simulink library "ammclib_bam_S32K3xx"  (R2016a)
(part 26 of 50)

      | text(tX,tY, 'AMCLIB_FluxEstimAB_FLT', 'horizontalAlignment', 'center');
      | if showStates == 2
      |   color('red');
      |   text(tX,tY - 20, ['debugging mode' char(13) char(10) '(limited performance)'], 'horizontalAlignment', 'center');
      | end
  AMCLIB_SpeedLoop_FLT : Subsystem  StartFcn=|  TreatAsAtomicUnit=on  mask(AMCLIB_SpeedLoop_FLT){showStates=Hide (faster execution), resetStatesEnable=Pre-set according to the first set of inputs after reset, showDebugOutputs=Hide, fltState_Out_showOutput=off, SampleTime=-1, wf0=30, wksi=1, J=1.6e-5, Kt=0.067, lambdaW=0.9, ramprpm=6, mechspeed=3000, polepairs=1, autoCalcEn=on, fltLambdaW=0, fltPropGainQ=0, fltIntegGainQ=0, fltLowerLimitQ=0, fltUpperLimitQ=0, fltRampUp=0, fltRampDown=0, SampleTime_1=NaN}
      | ts=get_param(gcb,'CompiledSampleTime');
      | if iscell(ts)
      |   ts=ts{1};
      |   if iscell(ts)
      |     ts=ts{1};
      |   end
      | end
      | ts=ts(1);
      | set_param(gcb,'SampleTime_1',num2str(ts));
      | p=Simulink.Mask.get(gcb);
      | hintText=p.getDialogControl('timeHint');
      | SampleTime=Simulink.data.evalinGlobal(bdroot,get_param(gcb,'SampleTime'));
      | p=Simulink.Mask.get(gcb);
      | autoCalcEn=get_param(gcb,'autoCalcEn');
      | if strcmp(autoCalcEn,'on')
      |   if SampleTime==-1
      |     hintText.Prompt='Caution: Implementation parameters depend on inherited sample time. Make sure that the sample time of the block''s inputs corresponds to the sampling period in the target application.';
      |   else
      |     hintText.Prompt='Caution: Implementation parameters depend on the sample time. Make sure that the simulation time step corresponds to the sampling period in the target application.';
      |   end
      |   SampleTime=ts;
      |   fltLambdaW_bkup=get_param(gcb,'fltLambdaW');
      |   fltPropGainQ_bkup=get_param(gcb,'fltPropGainQ');
      |   fltIntegGainQ_bkup=get_param(gcb,'fltIntegGainQ');
      |   fltLowerLimitQ_bkup=get_param(gcb,'fltLowerLimitQ');
      |   fltUpperLimitQ_bkup=get_param(gcb,'fltUpperLimitQ');
      |   fltRampUp_bkup=get_param(gcb,'fltRampUp');
      |   fltRampDown_bkup=get_param(gcb,'fltRampDown');
      |   wf0=Simulink.data.evalinGlobal(bdroot,get_param(gcb,'wf0'));
      |   wksi=Simulink.data.evalinGlobal(bdroot,get_param(gcb,'wksi'));
      |   J=Simulink.data.evalinGlobal(bdroot,get_param(gcb,'J'));
      |   Kt=Simulink.data.evalinGlobal(bdroot,get_param(gcb,'Kt'));
      |   lambdaW=Simulink.data.evalinGlobal(bdroot,get_param(gcb,'lambdaW'));
      |   ramprpm=Simulink.data.evalinGlobal(bdroot,get_param(gcb,'ramprpm'));
      |   mechspeed=Simulink.data.evalinGlobal(bdroot,get_param(gcb,'mechspeed'));
      |   polepairs=Simulink.data.evalinGlobal(bdroot,get_param(gcb,'polepairs'));
      |   if (wf0<=0)
      |     warning('Natural frequency f0 must be positive.');
      |   end
      |   if (wksi<=0)
      |     warning('Current loop attenuation must be positive.');
      |   end
      |   if (wksi>1)
      |     warning('Current loop attenuation must not exceed 1.');
      |   end
      |   if (J<=0)
      |     warning('Moment of inertia J must be positive.');
      |   end
      |   if (Kt<=0)
      |     warning('Torque constant Kt must be positive.');
      |   end
      |   if (lambdaW<0)
      |     warning('MA filter smoothing factor must be in the range 0..1.');
      |   end
      |   if (lambdaW>1)
      |     warning('MA filter smoothing factor must be in the range 0..1.');
      |   end
      |   if (mechspeed<=0)
      |     warning('Max. speed must be positive.');
      |   end
      |   if (polepairs<1)
      |     warning('Number of pole pairs must be a natural number (1, 2, 3, ...).');
      |   end
      |   if (round(polepairs)~=polepairs)
      |     warning('Number of pole pairs must be a natural number (1, 2, 3, ...).');
      |   end
      |   w0=6.283185307179586*wf0;
      |   pgain=2.0*wksi*w0*J/Kt;
      |   igain=w0*w0*J/Kt;
      |   wmax=polepairs*mechspeed*0.1047197551196598;
      |   fltPropGainQ=pgain;
      |   fltIntegGainQ=igain*SampleTime*0.5;
      |   fltLowerLimitQ=-wmax;
      |   fltUpperLimitQ=wmax;
      |   fltLambdaW=lambdaW;
      |   rampsc=polepairs*abs(ramprpm)*0.1047197551196598;
      |   fltRampUp=rampsc;
      |   fltRampDown=rampsc;
      |   if isnan(fltLambdaW)
      |     if ~strcmp(fltLambdaW_bkup,'0')
      |       set_param(gcb,'fltLambdaW','0');
      |     end
      |   else
      |     tmps=num2str(fltLambdaW);
      |     if ~strcmp(fltLambdaW_bkup,tmps)
      |       set_param(gcb,'fltLambdaW',tmps);
      |     end
      |   end
      |   if isnan(fltPropGainQ)
      |     if ~strcmp(fltPropGainQ_bkup,'0')
      |       set_param(gcb,'fltPropGainQ','0');
      |     end
      |   else
      |     tmps=num2str(fltPropGainQ);
      |     if ~strcmp(fltPropGainQ_bkup,tmps)
      |       set_param(gcb,'fltPropGainQ',tmps);
      |     end
      |   end
      |   if isnan(fltIntegGainQ)
      |     if ~strcmp(fltIntegGainQ_bkup,'0')
      |       set_param(gcb,'fltIntegGainQ','0');
      |     end
      |   else
      |     tmps=num2str(fltIntegGainQ);
      |     if ~strcmp(fltIntegGainQ_bkup,tmps)
      |       set_param(gcb,'fltIntegGainQ',tmps);
      |     end
      |   end
      |   if isnan(fltLowerLimitQ)
      |     if ~strcmp(fltLowerLimitQ_bkup,'0')
      |       set_param(gcb,'fltLowerLimitQ','0');
      |     end
      |   else
      |     tmps=num2str(fltLowerLimitQ);
      |     if ~strcmp(fltLowerLimitQ_bkup,tmps)
      |       set_param(gcb,'fltLowerLimitQ',tmps);
      |     end
      |   end
      |   if isnan(fltUpperLimitQ)
      |     if ~strcmp(fltUpperLimitQ_bkup,'0')
      |       set_param(gcb,'fltUpperLimitQ','0');
      |     end
      |   else
      |     tmps=num2str(fltUpperLimitQ);
      |     if ~strcmp(fltUpperLimitQ_bkup,tmps)
      |       set_param(gcb,'fltUpperLimitQ',tmps);
      |     end
      |   end
      |   if isnan(fltRampUp)
      |     if ~strcmp(fltRampUp_bkup,'0')
      |       set_param(gcb,'fltRampUp','0');
      |     end
      |   else
      |     tmps=num2str(fltRampUp);
      |     if ~strcmp(fltRampUp_bkup,tmps)
      |       set_param(gcb,'fltRampUp',tmps);
      |     end
      |   end
      |   if isnan(fltRampDown)
      |     if ~strcmp(fltRampDown_bkup,'0')
      |       set_param(gcb,'fltRampDown','0');
      |     end
      |   else
      |     tmps=num2str(fltRampDown);
      |     if ~strcmp(fltRampDown_bkup,tmps)
      |       set_param(gcb,'fltRampDown',tmps);
      |     end
      |   end
      | end
      mask prompts: showStates "Show internal states:"; resetStatesEnable "Internal state after reset:"; showDebugOutputs "Show debugging outputs:"; fltState_Out_showOutput "Output speed ramp state (fltState_Out)"; SampleTime "Sample time (-1 for inherited):"; wf0 "Speed loop natural frequency f0 [Hz]:"; wksi "Speed loop attenuation ξ:"; J "Moment of inertia J [kg*m^2]:"; Kt "Motor torque constant Kt [N*m/A]:"; lambdaW "Speed MA filter smoothing factor λ (0..1):"; ramprpm "Speed ramp slope [ΔRPM per speed loop iteration]:"; mechspeed "Maximum mechanical speed of the motor [RPM]:"; polepairs "Number of pole pairs of the motor:"; autoCalcEn "Calculate implementation parameters from physical parameters"; fltLambdaW "fltLambdaW (GDFLIB_FilterMA - smoothing factor):"; fltPropGainQ "fltPropGainQ (GFLIB_ControllerPIpAW - proportional gain):"; fltIntegGainQ "fltIntegGainQ (GFLIB_ControllerPIpAW - integral gain):"; fltLowerLimitQ "fltLowerLimitQ (GFLIB_ControllerPIpAW - lower limit):"; fltUpperLimitQ "fltUpperLimitQ (GFLIB_ControllerPIpAW - upper limit):"; fltRampUp "fltRampUp (Ramp up increment coefficient):"; fltRampDown "fltRampDown (Ramp decrement coefficient):"; SampleTime_1 "Discrete sample time:"
      mask help: Speed loop controller for the PMSM field-oriented control algorithm in single precision floating-point implementation. This block supports re-initialization of the internal state during simulation. If the block is reset, the outputs of the MA filter, PI controller, and the ramp will be aligned with the inputs fltFilterMAWOut_preset, fltControllerPIpAWQOut_preset, and fltRampOut_preset. Refer to the AMMCLIB User's Guide for further details.
      mask init:
      | ddName = get_param(bdroot,'DataDictionary');
      | if length(ddName)==0
      |   set_param(bdroot,'DataDictionary','ammclib_types.sldd');
      | else
      |   dd = Simulink.data.dictionary.open(ddName);
      |   data = getSection(dd,'Design Data');
      |   if ~exist(data,'SWLIBS_2Syst_F16')
      |     addDataSource(dd,'ammclib_types.sldd');
      |     saveChanges(dd);
      |   end
      | end
      | outputsChanged = 0;
      | 
      | if showStates == 1
      |   % hidden state variables
      |   if strcmp(get_param([gcb '/fltLambdaW'], 'BlockType'), 'Inport')
      |     posblk = get_param(gcb, 'Position');
      | 
      |     pos = get_param([gcb, '/fltLambdaW'], 'Position');
      |     orient = get_param([gcb, '/fltLambdaW'], 'Orientation');
      |     delete_block([gcb, '/fltLambdaW']);
      |     add_block('built-in/Ground', [gcb, '/fltLambdaW'], 'Position', pos, 'Orientation', orient);
      | 
      |     pos = get_param([gcb, '/fltPropGainQ'], 'Position');
      |     orient = get_param([gcb, '/fltPropGainQ'], 'Orientation');
      |     delete_block([gcb, '/fltPropGainQ']);
      |     add_block('built-in/Ground', [gcb, '/fltPropGainQ'], 'Position', pos, 'Orientation', orient);
      | 
      |     pos = get_param([gcb, '/fltIntegGainQ'], 'Position');
      |     orient = get_param([gcb, '/fltIntegGainQ'], 'Orientation');
      |     delete_block([gcb, '/fltIntegGainQ']);
      |     add_block('built-in/Ground', [gcb, '/fltIntegGainQ'], 'Position', pos, 'Orientation', orient);
      | 
      |     pos = get_param([gcb, '/fltLowerLimitQ'], 'Position');
      |     orient = get_param([gcb, '/fltLowerLimitQ'], 'Orientation');
      |     delete_block([gcb, '/fltLowerLimitQ']);
      |     add_block('built-in/Ground', [gcb, '/fltLowerLimitQ'], 'Position', pos, 'Orientation', orient);
      | 
      |     pos = get_param([gcb, '/fltUpperLimitQ'], 'Position');
      |     orient = get_param([gcb, '/fltUpperLimitQ'], 'Orientation');
      |     delete_block([gcb, '/fltUpperLimitQ']);
      |     add_block('built-in/Ground', [gcb, '/fltUpperLimitQ'], 'Position', pos, 'Orientation', orient);
      | 
      |     pos = get_param([gcb, '/fltRampUp'], 'Position');
      |     orient = get_param([gcb, '/fltRampUp'], 'Orientation');
      |     delete_block([gcb, '/fltRampUp']);
      |     add_block('built-in/Ground', [gcb, '/fltRampUp'], 'Position', pos, 'Orientation', orient);
      | 
      |     pos = get_param([gcb, '/fltRampDown'], 'Position');
      |     orient = get_param([gcb, '/fltRampDown'], 'Orientation');
      |     delete_block([gcb, '/fltRampDown']);
      |     add_block('built-in/Ground', [gcb, '/fltRampDown'], 'Position', pos, 'Orientation', orient);
      | 
      |     pos = get_param([gcb, '/fltAccW'], 'Position');
      |     orient = get_param([gcb, '/fltAccW'], 'Orientation');
      |     delete_block([gcb, '/fltAccW']);
      |     add_block('built-in/Ground', [gcb, '/fltAccW'], 'Position', pos, 'Orientation', orient);
      | 
      |     pos = get_param([gcb, '/fltIntegPartK_1Q'], 'Position');
      |     orient = get_param([gcb, '/fltIntegPartK_1Q'], 'Orientation');
      |     delete_block([gcb, '/fltIntegPartK_1Q']);
      |     add_block('built-in/Ground', [gcb, '/fltIntegPartK_1Q'], 'Position', pos, 'Orientation', orient);
      | 
      |     pos = get_param([gcb, '/fltInK_1Q'], 'Position');
      |     orient = get_param([gcb, '/fltInK_1Q'], 'Orientation');
      |     delete_block([gcb, '/fltInK_1Q']);
      |     add_block('built-in/Ground', [gcb, '/fltInK_1Q'], 'Position', pos, 'Orientation', orient);
      | 
      |     pos = get_param([gcb, '/fltState'], 'Position');
      |     orient = get_param([gcb, '/fltState'], 'Orientation');
      |     delete_block([gcb, '/fltState']);
      |     add_block('built-in/Ground', [gcb, '/fltState'], 'Position', pos, 'Orientation', orient);
      | 
      | 
      |     pmask=Simulink.Mask.get(gcb);
      |     pctrl=pmask.getParameter('SampleTime');
      |     pctrl.set('TypeOptions',{'fltVelocityReq/SampleTime','fltVelocityFbck/SampleTime','fltFilterMAWOut_preset/SampleTime','fltControllerPIpAWQOut_preset/SampleTime','fltRampOut_preset/SampleTime'});
      | 
      |     pos = get_param([gcb '/fltAccW_Out'], 'Position');
      |     orient = get_param([gcb '/fltAccW_Out'], 'Orientation');
      |     delete_block([gcb '/fltAccW_Out']);
      |     add_block('built-in/Terminator', [gcb '/fltAccW_Out'], 'Position', pos, 'Orientation', orient);
      | 
      |     pos = get_param([gcb '/fltIntegPartK_1Q_Out'], 'Position');
      |     orient = get_param([gcb '/fltIntegPartK_1Q_Out'], 'Orientation');
      |     delete_block([gcb '/fltIntegPartK_1Q_Out']);
      |     add_block('built-in/Terminator', [gcb '/fltIntegPartK_1Q_Out'], 'Position', pos, 'Orientation', orient);
      | 
      |     pos = get_param([gcb '/fltInK_1Q_Out'], 'Position');
      |     orient = get_param([gcb '/fltInK_1Q_Out'], 'Orientation');
      |     delete_block([gcb '/fltInK_1Q_Out']);
      |     add_block('built-in/Terminator', [gcb '/fltInK_1Q_Out'], 'Position', pos, 'Orientation', orient);
      | 
      |     if strcmp(get_param([gcb '/fltWReqFilt'], 'BlockType'), 'Outport')
      |       pos = get_param([gcb '/fltWReqFilt'], 'Position');
      |       orient = get_param([gcb '/fltWReqFilt'], 'Orientation');
      |       delete_block([gcb '/fltWReqFilt']);
      |       add_block('built-in/Terminator', [gcb '/fltWReqFilt'], 'Position', pos, 'Orientation', orient);
      | 
      |       pos = get_param([gcb '/fltWErr'], 'Position');
      |       orient = get_param([gcb '/fltWErr'], 'Orientation');
      |       delete_block([gcb '/fltWErr']);
      |       add_block('built-in/Terminator', [gcb '/fltWErr'], 'Position', pos, 'Orientation', orient);
      | 
      |       pos = get_param([gcb '/fltWFbckFilt'], 'Position');
      |       orient = get_param([gcb '/fltWFbckFilt'], 'Orientation');
      |       delete_block([gcb '/fltWFbckFilt']);
      |       add_block('built-in/Terminator', [gcb '/fltWFbckFilt'], 'Position', pos, 'Orientation', orient);
      | 
      |     end
      | 
      |     set_param([gcb '/fltVelocityReq'], 'Port', '1');
      |     set_param([gcb '/fltVelocityFbck'], 'Port', '2');
      |     set_param([gcb '/fltFilterMAWOut_preset'], 'Port', '3');
      |     set_param([gcb '/fltControllerPIpAWQOut_preset'], 'Port', '4');
      |     set_param([gcb '/fltRampOut_preset'], 'Port', '5');
      | 
      |     tmpOutCnt=0;
      |     tmpOutCnt=tmpOutCnt+1;
      |     set_param([gcb '/pIDQReq'], 'Port', num2str(tmpOutCnt));
      |     tmpOutCnt=tmpOutCnt+1;
      |     set_param([gcb '/u16LimitFlagQ'], 'Port', num2str(tmpOutCnt));
      |     if strcmp(get_param([gcb '/fltState_Out'], 'BlockType'), 'Outport')
      |       tmpOutCnt=tmpOutCnt+1;
      |       set_param([gcb '/fltState_Out'], 'Port', num2str(tmpOutCnt));
      |     end
      | 
      |   autoCalcEn=get_param(gcb,'autoCalcEn');
      |   if strcmp(autoCalcEn,'on')
      |     set_param(gcb,'MaskEnables',{'on','on','off','on','on','on','on','on','on','on','on','on','on','on','on','on','on','on','on','on','on','off'});
      |   else
      |     set_param(gcb,'MaskEnables',{'on','on','off','on','on','off','off','off','off','off','off','off','off','on','on','on','on','on','on','on','on','off'});
      |   end
      | 
      |     if (posblk(4) - posblk(2)) > 150
      |       height = 150;
      |       set_param(gcb,'Position',[posblk(1), posblk(2), posblk(3), posblk(2)+height])
      |     end
      |   end
      | else
      |   % shown state variables
      |   if strcmp(get_param([gcb '/fltLambdaW'], 'BlockType'), 'Ground')
      |     posblk = get_param(gcb, 'Position');
      | 
      |     pos = get_param([gcb, '/fltLambdaW'], 'Position');
      |     orient = get_param([gcb, '/fltLambdaW'], 'Orientation');
      |     delete_block([gcb, '/fltLambdaW']);
      |     add_block('built-in/Inport', [gcb, '/fltLambdaW'], 'Position', pos, 'Orientation', orient, 'OutDataTypeStr', 'single');
      | 
      |     pos = get_param([gcb, '/fltPropGainQ'], 'Position');
      |     orient = get_param([gcb, '/fltPropGainQ'], 'Orientation');
      |     delete_block([gcb, '/fltPropGainQ']);
      |     add_block('built-in/Inport', [gcb, '/fltPropGainQ'], 'Position', pos, 'Orientation', orient, 'OutDataTypeStr', 'single');
      | 
      |     pos = get_param([gcb, '/fltIntegGainQ'], 'Position');
      |     orient = get_param([gcb, '/fltIntegGainQ'], 'Orientation');
      |     delete_block([gcb, '/fltIntegGainQ']);
      |     add_block('built-in/Inport', [gcb, '/fltIntegGainQ'], 'Position', pos, 'Orientation', orient, 'OutDataTypeStr', 'single');
      | 
      |     pos = get_param([gcb, '/fltLowerLimitQ'], 'Position');
      |     orient = get_param([gcb, '/fltLowerLimitQ'], 'Orientation');
      |     delete_block([gcb, '/fltLowerLimitQ']);
      |     add_block('built-in/Inport', [gcb, '/fltLowerLimitQ'], 'Position', pos, 'Orientation', orient, 'OutDataTypeStr', 'single');
      | 
      |     pos = get_param([gcb, '/fltUpperLimitQ'], 'Position');
      |     orient = get_param([gcb, '/fltUpperLimitQ'], 'Orientation');
      |     delete_block([gcb, '/fltUpperLimitQ']);
      |     add_block('built-in/Inport', [gcb, '/fltUpperLimitQ'], 'Position', pos, 'Orientation', orient, 'OutDataTypeStr', 'single');
      | 
      |     pos = get_param([gcb, '/fltRampUp'], 'Position');
      |     orient = get_param([gcb, '/fltRampUp'], 'Orientation');
      |     delete_block([gcb, '/fltRampUp']);
      |     add_block('built-in/Inport', [gcb, '/fltRampUp'], 'Position', pos, 'Orientation', orient, 'OutDataTypeStr', 'single');
      | 
      |     pos = get_param([gcb, '/fltRampDown'], 'Position');
      |     orient = get_param([gcb, '/fltRampDown'], 'Orientation');
      |     delete_block([gcb, '/fltRampDown']);
      |     add_block('built-in/Inport', [gcb, '/fltRampDown'], 'Position', pos, 'Orientation', orient, 'OutDataTypeStr', 'single');
      | 
      |     pos = get_param([gcb, '/fltAccW'], 'Position');
      |     orient = get_param([gcb, '/fltAccW'], 'Orientation');
      |     delete_block([gcb, '/fltAccW']);
      |     add_block('built-in/Inport', [gcb, '/fltAccW'], 'Position', pos, 'Orientation', orient, 'OutDataTypeStr', 'single');
      | 
      |     pos = get_param([gcb, '/fltIntegPartK_1Q'], 'Position');
      |     orient = get_param([gcb, '/fltIntegPartK_1Q'], 'Orientation');
      |     delete_block([gcb, '/fltIntegPartK_1Q']);
      |     add_block('built-in/Inport', [gcb, '/fltIntegPartK_1Q'], 'Position', pos, 'Orientation', orient, 'OutDataTypeStr', 'single');
      | 
      |     pos = get_param([gcb, '/fltInK_1Q'], 'Position');
      |     orient = get_param([gcb, '/fltInK_1Q'], 'Orientation');
      |     delete_block([gcb, '/fltInK_1Q']);
      |     add_block('built-in/Inport', [gcb, '/fltInK_1Q'], 'Position', pos, 'Orientation', orient, 'OutDataTypeStr', 'single');
      | 
      |     pos = get_param([gcb, '/fltState'], 'Position');
      |     orient = get_param([gcb, '/fltState'], 'Orientation');
      |     delete_block([gcb, '/fltState']);
      |     add_block('built-in/Inport', [gcb, '/fltState'], 'Position', pos, 'Orientation', orient, 'OutDataTypeStr', 'single');
      | 
      | 
      | 
      |     pos = get_param([gcb '/fltAccW_Out'], 'Position');
      |     orient = get_param([gcb '/fltAccW_Out'], 'Orientation');
      |     delete_block([gcb '/fltAccW_Out']);
      |     add_block('built-in/Outport', [gcb '/fltAccW_Out'], 'Position', pos, 'Orientation', orient);
      | 
      |     pos = get_param([gcb '/fltIntegPartK_1Q_Out'], 'Position');
      |     orient = get_param([gcb '/fltIntegPartK_1Q_Out'], 'Orientation');
      |     delete_block([gcb '/fltIntegPartK_1Q_Out']);
      |     add_block('built-in/Outport', [gcb '/fltIntegPartK_1Q_Out'], 'Position', pos, 'Orientation', orient);
      | 
      |     pos = get_param([gcb '/fltInK_1Q_Out'], 'Position');
      |     orient = get_param([gcb '/fltInK_1Q_Out'], 'Orientation');
      |     delete_block([gcb '/fltInK_1Q_Out']);
      |     add_block('built-in/Outport', [gcb '/fltInK_1Q_Out'], 'Position', pos, 'Orientation', orient);
      | 
      | 
      |     pmask=Simulink.Mask.get(gcb);
      |     pctrl=pmask.getParameter('SampleTime');
      |     pctrl.set('TypeOptions',{'fltVelocityReq/SampleTime','fltVelocityFbck/SampleTime','fltFilterMAWOut_preset/SampleTime','fltControllerPIpAWQOut_preset/SampleTime','fltRampOut_preset/SampleTime','fltLambdaW/SampleTime','fltPropGainQ/SampleTime','fltIntegGainQ/SampleTime','fltLowerLimitQ/SampleTime','fltUpperLimitQ/SampleTime','fltRampUp/SampleTime','fltRampDown/SampleTime','fltAccW/SampleTime','fltIntegPartK_1Q/SampleTime','fltInK_1Q/SampleTime','fltState/SampleTime'});
      | 
      |     if (showDebugOutputs == 2) && (strcmp(get_param([gcb '/fltWReqFilt'], 'BlockType'), 'Terminator'))
      |       pos = get_param([gcb '/fltWReqFilt'], 'Position');
      |       orient = get_param([gcb '/fltWReqFilt'], 'Orientation');
      |       delete_block([gcb '/fltWReqFilt']);
      |       add_block('built-in/Outport', [gcb '/fltWReqFilt'], 'Position', pos, 'Orientation', orient);
      | 
      |       pos = get_param([gcb '/fltWErr'], 'Position');
      |       orient = get_param([gcb '/fltWErr'], 'Orientation');
      |       delete_block([gcb '/fltWErr']);
      |       add_block('built-in/Outport', [gcb '/fltWErr'], 'Position', pos, 'Orientation', orient);
      | 
      |       pos = get_param([gcb '/fltWFbckFilt'], 'Position');
      |       orient = get_param([gcb '/fltWFbckFilt'], 'Orientation');
      |       delete_block([gcb '/fltWFbckFilt']);
      |       add_block('built-in/Outport', [gcb '/fltWFbckFilt'], 'Position', pos, 'Orientation', orient);
      | 
      |     end
      | 
      |     set_param([gcb '/fltVelocityReq'], 'Port', '1');
      |     set_param([gcb '/fltVelocityFbck'], 'Port', '2');
      |     set_param([gcb '/fltFilterMAWOut_preset'], 'Port', '3');
      |     set_param([gcb '/fltControllerPIpAWQOut_preset'], 'Port', '4');
      |     set_param([gcb '/fltRampOut_preset'], 'Port', '5');
      |     set_param([gcb '/fltLambdaW'], 'Port', '6');
      |     set_param([gcb '/fltPropGainQ'], 'Port', '7');
      |     set_param([gcb '/fltIntegGainQ'], 'Port', '8');
      |     set_param([gcb '/fltLowerLimitQ'], 'Port', '9');
      |     set_param([gcb '/fltUpperLimitQ'], 'Port', '10');
      |     set_param([gcb '/fltRampUp'], 'Port', '11');
      |     set_param([gcb '/fltRampDown'], 'Port', '12');
      |     set_param([gcb '/fltAccW'], 'Port', '13');
      |     set_param([gcb '/fltIntegPartK_1Q'], 'Port', '14');
      |     set_param([gcb '/fltInK_1Q'], 'Port', '15');
      |     set_param([gcb '/fltState'], 'Port', '16');
      | 
      |     if (showDebugOutputs == 2)
      |       tmpOutCnt=0;
      |       tmpOutCnt=tmpOutCnt+1;
      |       set_param([gcb '/pIDQReq'], 'Port', num2str(tmpOutCnt));
      |       tmpOutCnt=tmpOutCnt+1;
      |       set_param([gcb '/u16LimitFlagQ'], 'Port', num2str(tmpOutCnt));
      |       tmpOutCnt=tmpOutCnt+1;
      |       set_param([gcb '/fltWReqFilt'], 'Port', num2str(tmpOutCnt));
      |       tmpOutCnt=tmpOutCnt+1;
      |       set_param([gcb '/fltWErr'], 'Port', num2str(tmpOutCnt));
      |       tmpOutCnt=tmpOutCnt+1;
      |       set_param([gcb '/fltWFbckFilt'], 'Port', num2str(tmpOutCnt));
      |       tmpOutCnt=tmpOutCnt+1;
      |       set_param([gcb '/fltAccW_Out'], 'Port', num2str(tmpOutCnt));
      |       tmpOutCnt=tmpOutCnt+1;
      |       set_param([gcb '/fltIntegPartK_1Q_Out'], 'Port', num2str(tmpOutCnt));
      |       tmpOutCnt=tmpOutCnt+1;
      |       set_param([gcb '/fltInK_1Q_Out'], 'Port', num2str(tmpOutCnt));
      |       if strcmp(get_param([gcb '/fltState_Out'], 'BlockType'), 'Outport')
      |         tmpOutCnt=tmpOutCnt+1;
      |         set_param([gcb '/fltState_Out'], 'Port', num2str(tmpOutCnt));
      |       end
      |     else
      |       tmpOutCnt=0;
      |       tmpOutCnt=tmpOutCnt+1;
      |       set_param([gcb '/pIDQReq'], 'Port', num2str(tmpOutCnt));
      |       tmpOutCnt=tmpOutCnt+1;
      |       set_param([gcb '/u16LimitFlagQ'], 'Port', num2str(tmpOutCnt));
      |       tmpOutCnt=tmpOutCnt+1;
      |       set_param([gcb '/fltAccW_Out'], 'Port', num2str(tmpOutCnt));
      |       tmpOutCnt=tmpOutCnt+1;
      |       set_param([gcb '/fltIntegPartK_1Q_Out'], 'Port', num2str(tmpOutCnt));
      |       tmpOutCnt=tmpOutCnt+1;
      |       set_param([gcb '/fltInK_1Q_Out'], 'Port', num2str(tmpOutCnt));
      |       if strcmp(get_param([gcb '/fltState_Out'], 'BlockType'), 'Outport')
      |         tmpOutCnt=tmpOutCnt+1;
      |         set_param([gcb '/fltState_Out'], 'Port', num2str(tmpOutCnt));
      |       end
      |     end
      | 
      |     set_param(gcb,'MaskEnables',{'on','on','on','on','on','off','off','off','off','off','off','off','off','off','off','off','off','off','off','off','off','off'});
      | 
      |     if (posblk(4) - posblk(2)) < 425
      |       height = 425;
      |       set_param(gcb,'Position',[posblk(1), posblk(2), posblk(3), posblk(2)+height])
      |     end
      |   else
      |     if (showDebugOutputs == 2) && (strcmp(get_param([gcb '/fltWReqFilt'], 'BlockType'), 'Terminator'))
      |       % shown debugging outputs
      |       pos = get_param([gcb '/fltWReqFilt'], 'Position');
      |       orient = get_param([gcb '/fltWReqFilt'], 'Orientation');
      |       delete_block([gcb '/fltWReqFilt']);
      |       add_block('built-in/Outport', [gcb '/fltWReqFilt'], 'Position', pos, 'Orientation', orient);
      | 
      |       pos = get_param([gcb '/fltWErr'], 'Position');
      |       orient = get_param([gcb '/fltWErr'], 'Orientation');
      |       delete_block([gcb '/fltWErr']);
      |       add_block('built-in/Outport', [gcb '/fltWErr'], 'Position', pos, 'Orientation', orient);
      | 
      |       pos = get_param([gcb '/fltWFbckFilt'], 'Position');
      |       orient = get_param([gcb '/fltWFbckFilt'], 'Orientation');
      |       delete_block([gcb '/fltWFbckFilt']);
      |       add_block('built-in/Outport', [gcb '/fltWFbckFilt'], 'Position', pos, 'Orientation', orient);
      | 
      |       tmpOutCnt=0;
      |       tmpOutCnt=tmpOutCnt+1;
      |       set_param([gcb '/pIDQReq'], 'Port', num2str(tmpOutCnt));
      |       tmpOutCnt=tmpOutCnt+1;
      |       set_param([gcb '/u16LimitFlagQ'], 'Port', num2str(tmpOutCnt));
      |       tmpOutCnt=tmpOutCnt+1;
      |       set_param([gcb '/fltWReqFilt'], 'Port', num2str(tmpOutCnt));
      |       tmpOutCnt=tmpOutCnt+1;
      |       set_param([gcb '/fltWErr'], 'Port', num2str(tmpOutCnt));
      |       tmpOutCnt=tmpOutCnt+1;
      |       set_param([gcb '/fltWFbckFilt'], 'Port', num2str(tmpOutCnt));
      |       tmpOutCnt=tmpOutCnt+1;
      |       set_param([gcb '/fltAccW_Out'], 'Port', num2str(tmpOutCnt));
      |       tmpOutCnt=tmpOutCnt+1;
      |       set_param([gcb '/fltIntegPartK_1Q_Out'], 'Port', num2str(tmpOutCnt));
      |       tmpOutCnt=tmpOutCnt+1;
      |       set_param([gcb '/fltInK_1Q_Out'], 'Port', num2str(tmpOutCnt));
      |       if strcmp(get_param([gcb '/fltState_Out'], 'BlockType'), 'Outport')
      |         tmpOutCnt=tmpOutCnt+1;
      |         set_param([gcb '/fltState_Out'], 'Port', num2str(tmpOutCnt));
      |       end
      |     elseif (showDebugOutputs == 1) && (strcmp(get_param([gcb '/fltWReqFilt'], 'BlockType'), 'Outport'))
      |       % hidden debugging outputs
      |       pos = get_param([gcb '/fltWReqFilt'], 'Position');
      |       orient = get_param([gcb '/fltWReqFilt'], 'Orientation');
      |       delete_block([gcb '/fltWReqFilt']);
      |       add_block('built-in/Terminator', [gcb '/fltWReqFilt'], 'Position', pos, 'Orientation', orient);
      | 
      |       pos = get_param([gcb '/fltWErr'], 'Position');
      |       orient = get_param([gcb '/fltWErr'], 'Orientation');
      |       delete_block([gcb '/fltWErr']);
      |       add_block('built-in/Terminator', [gcb '/fltWErr'], 'Position', pos, 'Orientation', orient);
      | 
      |       pos = get_param([gcb '/fltWFbckFilt'], 'Position');
      |       orient = get_param([gcb '/fltWFbckFilt'], 'Orientation');
      |       delete_block([gcb '/fltWFbckFilt']);
      |       add_block('built-in/Terminator', [gcb '/fltWFbckFilt'], 'Position', pos, 'Orientation', orient);
      | 
      |       tmpOutCnt=0;
      |       tmpOutCnt=tmpOutCnt+1;
      |       set_param([gcb '/pIDQReq'], 'Port', num2str(tmpOutCnt));
      |       tmpOutCnt=tmpOutCnt+1;
      |       set_param([gcb '/u16LimitFlagQ'], 'Port', num2str(tmpOutCnt));
      |       tmpOutCnt=tmpOutCnt+1;
      |       set_param([gcb '/fltAccW_Out'], 'Port', num2str(tmpOutCnt));
      |       tmpOutCnt=tmpOutCnt+1;
      |       set_param([gcb '/fltIntegPartK_1Q_Out'], 'Port', num2str(tmpOutCnt));
      |       tmpOutCnt=tmpOutCnt+1;
      |       set_param([gcb '/fltInK_1Q_Out'], 'Port', num2str(tmpOutCnt));
      |       if strcmp(get_param([gcb '/fltState_Out'], 'BlockType'), 'Outport')
      |         tmpOutCnt=tmpOutCnt+1;
      |         set_param([gcb '/fltState_Out'], 'Port', num2str(tmpOutCnt));
      |       end
      |     end
      |   end
      | end
      | if strcmp(get_param(gcb,'fltState_Out_showOutput'),'on')
      |   if strcmp(get_param([gcb '/fltState_Out'], 'BlockType'), 'Terminator')
      |     pos = get_param([gcb '/fltState_Out'], 'Position');
      |     orient = get_param([gcb '/fltState_Out'], 'Orientation');
      |     delete_block([gcb '/fltState_Out']);
      |     add_block('built-in/Outport', [gcb '/fltState_Out'], 'Position', pos, 'Orientation', orient);
      |     outputsChanged = 1;
      |   end
      | else
      |   if strcmp(get_param([gcb '/fltState_Out'], 'BlockType'), 'Outport')
      |     pos = get_param([gcb '/fltState_Out'], 'Position');
      |     orient = get_param([gcb '/fltState_Out'], 'Orientation');
      |     delete_block([gcb '/fltState_Out']);
      |     add_block('built-in/Terminator', [gcb '/fltState_Out'], 'Position', pos, 'Orientation', orient);
      |     outputsChanged = 1;
      |   end
      | end
      | if outputsChanged == 1;
      |   tmpOutCnt = 0;
      |   if strcmp(get_param([gcb '/pIDQReq'], 'BlockType'), 'Outport')
      |     tmpOutCnt = tmpOutCnt + 1;
      |     set_param([gcb '/pIDQReq'], 'Port', num2str(tmpOutCnt));
      |   end
      |   if strcmp(get_param([gcb '/u16LimitFlagQ'], 'BlockType'), 'Outport')
      |     tmpOutCnt = tmpOutCnt + 1;
      |     set_param([gcb '/u16LimitFlagQ'], 'Port', num2str(tmpOutCnt));
      |   end
      |   if strcmp(get_param([gcb '/fltWReqFilt'], 'BlockType'), 'Outport')
      |     tmpOutCnt = tmpOutCnt + 1;
      |     set_param([gcb '/fltWReqFilt'], 'Port', num2str(tmpOutCnt));
      |   end
      |   if strcmp(get_param([gcb '/fltWErr'], 'BlockType'), 'Outport')
      |     tmpOutCnt = tmpOutCnt + 1;
      |     set_param([gcb '/fltWErr'], 'Port', num2str(tmpOutCnt));
      |   end
      |   if strcmp(get_param([gcb '/fltWFbckFilt'], 'BlockType'), 'Outport')
      |     tmpOutCnt = tmpOutCnt + 1;
      |     set_param([gcb '/fltWFbckFilt'], 'Port', num2str(tmpOutCnt));
      |   end
      |   if strcmp(get_param([gcb '/fltAccW_Out'], 'BlockType'), 'Outport')
      |     tmpOutCnt = tmpOutCnt + 1;
      |     set_param([gcb '/fltAccW_Out'], 'Port', num2str(tmpOutCnt));
      |   end
      |   if strcmp(get_param([gcb '/fltIntegPartK_1Q_Out'], 'BlockType'), 'Outport')
      |     tmpOutCnt = tmpOutCnt + 1;
      |     set_param([gcb '/fltIntegPartK_1Q_Out'], 'Port', num2str(tmpOutCnt));
      |   end
      |   if strcmp(get_param([gcb '/fltInK_1Q_Out'], 'BlockType'), 'Outport')
      |     tmpOutCnt = tmpOutCnt + 1;
      |     set_param([gcb '/fltInK_1Q_Out'], 'Port', num2str(tmpOutCnt));
      |   end
      |   if strcmp(get_param([gcb '/fltState_Out'], 'BlockType'), 'Outport')
      |     tmpOutCnt = tmpOutCnt + 1;
      |     set_param([gcb '/fltState_Out'], 'Port', num2str(tmpOutCnt));
      |   end
      | end
      settings: RTWSystemCode=Inline
      mask Help: web([fileparts(which('ammclib_bam_S32K3xx.slx')) '/../doc/S32K3XXMCLUG.pdf'], '-browser')
      mask TypeOptions showStates: Hide (faster execution) | Show (allows debugging; connect feedback loops manually)
      mask Callback showStates:
      | maskStr=get_param(gcb,'showStates');
      | if strcmp(maskStr,'Hide (faster execution)')
      |   autoCalcEn=get_param(gcb,'autoCalcEn');
      |   if strcmp(autoCalcEn,'on')
      |     set_param(gcb,'MaskEnables',{'on','on','off','on','on','on','on','on','on','on','on','on','on','on','on','on','on','on','on','on','on','off'});
      |   else
      |     set_param(gcb,'MaskEnables',{'on','on','off','on','on','off','off','off','off','off','off','off','off','on','on','on','on','on','on','on','on','off'});
      |   end
      | else
      |   set_param(gcb,'MaskEnables',{'on','on','on','on','on','off','off','off','off','off','off','off','off','off','off','off','off','off','off','off','off','off'});
      | end
      mask TypeOptions resetStatesEnable: Pre-set according to the first set of inputs after reset | Clear to zero
      mask TypeOptions showDebugOutputs: Hide | Show
      mask TypeOptions SampleTime: fltVelocityReq/SampleTime | fltVelocityFbck/SampleTime | fltFilterMAWOut_preset/SampleTime | fltControllerPIpAWQOut_preset/SampleTime | fltRampOut_preset/SampleTime
      mask Callback SampleTime:
      | p=Simulink.Mask.get(gcb);
      | hintText=p.getDialogControl('timeHint');
      | SampleTime=Simulink.data.evalinGlobal(bdroot,get_param(gcb,'SampleTime'));
      | SampleTime_1=str2double(get_param(gcb,'SampleTime_1'));
      | if (((SampleTime==-1) && (~contains(hintText.Prompt,'inherited'))) || ...
      |     ((SampleTime~=-1) && contains(hintText.Prompt,'inherited')) || ...
      |     ((SampleTime~=-1) && (SampleTime_1~=SampleTime)) || ...
      |     ((SampleTime_1~=-1) && contains(hintText.Prompt,'yet')))
      |   if ((SampleTime==-1) && (~contains(hintText.Prompt,'inherited')))
      |     set_param(gcb,'SampleTime_1',num2str(NaN));
      |     SampleTime_1=NaN;
      |   end
      |   if (SampleTime~=-1)
      |     set_param(gcb,'SampleTime_1',num2str(SampleTime));
      |     SampleTime_1=SampleTime;
      |   end
      |   autoCalcEn=get_param(gcb,'autoCalcEn');
      |   if strcmp(autoCalcEn,'on')
      |     p=Simulink.Mask.get(gcb);
      |     hintText=p.getDialogControl('timeHint');
      |     if SampleTime==-1
      |       SampleTime=SampleTime_1;
      |       if isnan(SampleTime)
      |         hintText.Prompt='Note: Implementation parameters cannot be calculated yet because the block''s inherited sample time is unknown. Simulink will update the sample time when you run the simulation.';
      |       else
      |         hintText.Prompt='Caution: Implementation parameters depend on inherited sample time. Make sure that the sample time of the block''s inputs corresponds to the sampling period in the target application.';
      |       end
      |     else
      |       hintText.Prompt='Caution: Implementation parameters depend on the sample time. Make sure that the simulation time step corresponds to the sampling period in the target application.';
      |     end
      |     fltLambdaW_bkup=get_param(gcb,'fltLambdaW');
      |     fltPropGainQ_bkup=get_param(gcb,'fltPropGainQ');
      |     fltIntegGainQ_bkup=get_param(gcb,'fltIntegGainQ');
      |     fltLowerLimitQ_bkup=get_param(gcb,'fltLowerLimitQ');
      |     fltUpperLimitQ_bkup=get_param(gcb,'fltUpperLimitQ');
      |     fltRampUp_bkup=get_param(gcb,'fltRampUp');
      |     fltRampDown_bkup=get_param(gcb,'fltRampDown');
      |     wf0=Simulink.data.evalinGlobal(bdroot,get_param(gcb,'wf0'));
      |     wksi=Simulink.data.evalinGlobal(bdroot,get_param(gcb,'wksi'));
      |     J=Simulink.data.evalinGlobal(bdroot,get_param(gcb,'J'));
      |     Kt=Simulink.data.evalinGlobal(bdroot,get_param(gcb,'Kt'));
      |     lambdaW=Simulink.data.evalinGlobal(bdroot,get_param(gcb,'lambdaW'));
      |     ramprpm=Simulink.data.evalinGlobal(bdroot,get_param(gcb,'ramprpm'));
      |     mechspeed=Simulink.data.evalinGlobal(bdroot,get_param(gcb,'mechspeed'));
      |     polepairs=Simulink.data.evalinGlobal(bdroot,get_param(gcb,'polepairs'));
      |     if (wf0<=0)
      |       warning('Natural frequency f0 must be positive.');
      |     end
      |     if (wksi<=0)
      |       warning('Current loop attenuation must be positive.');
      |     end
      |     if (wksi>1)
      |       warning('Current loop attenuation must not exceed 1.');
      |     end
      |     if (J<=0)
      |       warning('Moment of inertia J must be positive.');
      |     end
      |     if (Kt<=0)
      |       warning('Torque constant Kt must be positive.');
      |     end
      |     if (lambdaW<0)
      |       warning('MA filter smoothing factor must be in the range 0..1.');
      |     end
      |     if (lambdaW>1)
      |       warning('MA filter smoothing factor must be in the range 0..1.');
      |     end
      |     if (mechspeed<=0)
      |       warning('Max. speed must be positive.');
      |     end
      |     if (polepairs<1)
      |       warning('Number of pole pairs must be a natural number (1, 2, 3, ...).');
      |     end
      |     if (round(polepairs)~=polepairs)
      |       warning('Number of pole pairs must be a natural number (1, 2, 3, ...).');
      |     end
      |     w0=6.283185307179586*wf0;
      |     pgain=2.0*wksi*w0*J/Kt;
      |     igain=w0*w0*J/Kt;
      |     wmax=polepairs*mechspeed*0.1047197551196598;
      |     fltPropGainQ=pgain;
      |     fltIntegGainQ=igain*SampleTime*0.5;
      |     fltLowerLimitQ=-wmax;
      |     fltUpperLimitQ=wmax;
      |     fltLambdaW=lambdaW;
      |     rampsc=polepairs*abs(ramprpm)*0.1047197551196598;
      |     fltRampUp=rampsc;
      |     fltRampDown=rampsc;
      |     if isnan(fltLambdaW)
      |       if ~strcmp(fltLambdaW_bkup,'0')
      |         set_param(gcb,'fltLambdaW','0');
      |       end
      |     else
      |       tmps=num2str(fltLambdaW);
      |       if ~strcmp(fltLambdaW_bkup,tmps)
      |         set_param(gcb,'fltLambdaW',tmps);
      |       end
      |     end
      |     if isnan(fltPropGainQ)
      |       if ~strcmp(fltPropGainQ_bkup,'0')
      |         set_param(gcb,'fltPropGainQ','0');
      |       end
      |     else
      |       tmps=num2str(fltPropGainQ);
      |       if ~strcmp(fltPropGainQ_bkup,tmps)
      |         set_param(gcb,'fltPropGainQ',tmps);
      |       end
      |     end
      |     if isnan(fltIntegGainQ)
      |       if ~strcmp(fltIntegGainQ_bkup,'0')
      |         set_param(gcb,'fltIntegGainQ','0');
      |       end
      |     else
      |       tmps=num2str(fltIntegGainQ);
      |       if ~strcmp(fltIntegGainQ_bkup,tmps)
      |         set_param(gcb,'fltIntegGainQ',tmps);
      |       end
      |     end
      |     if isnan(fltLowerLimitQ)
      |       if ~strcmp(fltLowerLimitQ_bkup,'0')
      |         set_param(gcb,'fltLowerLimitQ','0');
      |       end
      |     else
      |       tmps=num2str(fltLowerLimitQ);
      |       if ~strcmp(fltLowerLimitQ_bkup,tmps)
      |         set_param(gcb,'fltLowerLimitQ',tmps);
      |       end
      |     end
      |     if isnan(fltUpperLimitQ)
      |       if ~strcmp(fltUpperLimitQ_bkup,'0')
      |         set_param(gcb,'fltUpperLimitQ','0');
      |       end
      |     else
      |       tmps=num2str(fltUpperLimitQ);
      |       if ~strcmp(fltUpperLimitQ_bkup,tmps)
      |         set_param(gcb,'fltUpperLimitQ',tmps);
      |       end
      |     end
      |     if isnan(fltRampUp)
      |       if ~strcmp(fltRampUp_bkup,'0')
      |         set_param(gcb,'fltRampUp','0');
      |       end
      |     else
      |       tmps=num2str(fltRampUp);
      |       if ~strcmp(fltRampUp_bkup,tmps)
      |         set_param(gcb,'fltRampUp',tmps);
      |       end
      |     end
      |     if isnan(fltRampDown)
      |       if ~strcmp(fltRampDown_bkup,'0')
      |         set_param(gcb,'fltRampDown','0');
      |       end
      |     else
      |       tmps=num2str(fltRampDown);
      |       if ~strcmp(fltRampDown_bkup,tmps)
      |         set_param(gcb,'fltRampDown',tmps);
      |       end
      |     end
      |   end
      | end
      mask Callback wf0:
      | autoCalcEn=get_param(gcb,'autoCalcEn');
      | if strcmp(autoCalcEn,'on')
      |   SampleTime=Simulink.data.evalinGlobal(bdroot,get_param(gcb,'SampleTime'));
      |   if (SampleTime==-1)
      |     SampleTime=str2double(get_param(gcb,'SampleTime_1'));
      |   end
      |   fltLambdaW_bkup=get_param(gcb,'fltLambdaW');
      |   fltPropGainQ_bkup=get_param(gcb,'fltPropGainQ');
      |   fltIntegGainQ_bkup=get_param(gcb,'fltIntegGainQ');
      |   fltLowerLimitQ_bkup=get_param(gcb,'fltLowerLimitQ');
      |   fltUpperLimitQ_bkup=get_param(gcb,'fltUpperLimitQ');
      |   fltRampUp_bkup=get_param(gcb,'fltRampUp');
      |   fltRampDown_bkup=get_param(gcb,'fltRampDown');
      |   wf0=Simulink.data.evalinGlobal(bdroot,get_param(gcb,'wf0'));
      |   wksi=Simulink.data.evalinGlobal(bdroot,get_param(gcb,'wksi'));
      |   J=Simulink.data.evalinGlobal(bdroot,get_param(gcb,'J'));
      |   Kt=Simulink.data.evalinGlobal(bdroot,get_param(gcb,'Kt'));
      |   lambdaW=Simulink.data.evalinGlobal(bdroot,get_param(gcb,'lambdaW'));
      |   ramprpm=Simulink.data.evalinGlobal(bdroot,get_param(gcb,'ramprpm'));
      |   mechspeed=Simulink.data.evalinGlobal(bdroot,get_param(gcb,'mechspeed'));
      |   polepairs=Simulink.data.evalinGlobal(bdroot,get_param(gcb,'polepairs'));
      |   if (wf0<=0)
      |     warning('Natural frequency f0 must be positive.');
      |   end
      |   if (wksi<=0)
      |     warning('Current loop attenuation must be positive.');
      |   end
      |   if (wksi>1)
      |     warning('Current loop attenuation must not exceed 1.');
      |   end
      |   if (J<=0)
      |     warning('Moment of inertia J must be positive.');
      |   end
      |   if (Kt<=0)
      |     warning('Torque constant Kt must be positive.');
      |   end
      |   if (lambdaW<0)
      |     warning('MA filter smoothing factor must be in the range 0..1.');
      |   end
      |   if (lambdaW>1)
      |     warning('MA filter smoothing factor must be in the range 0..1.');
      |   end
      |   if (mechspeed<=0)
      |     warning('Max. speed must be positive.');
      |   end
      |   if (polepairs<1)
      |     warning('Number of pole pairs must be a natural number (1, 2, 3, ...).');
      |   end
      |   if (round(polepairs)~=polepairs)
      |     warning('Number of pole pairs must be a natural number (1, 2, 3, ...).');
      |   end
      |   w0=6.283185307179586*wf0;
      |   pgain=2.0*wksi*w0*J/Kt;
      |   igain=w0*w0*J/Kt;
      |   wmax=polepairs*mechspeed*0.1047197551196598;
      |   fltPropGainQ=pgain;
      |   fltIntegGainQ=igain*SampleTime*0.5;
      |   fltLowerLimitQ=-wmax;
      |   fltUpperLimitQ=wmax;
      |   fltLambdaW=lambdaW;
      |   rampsc=polepairs*abs(ramprpm)*0.1047197551196598;
      |   fltRampUp=rampsc;
      |   fltRampDown=rampsc;
      |   if isnan(fltLambdaW)
      |     if ~strcmp(fltLambdaW_bkup,'0')
      |       set_param(gcb,'fltLambdaW','0');
      |     end
      |   else
      |     tmps=num2str(fltLambdaW);
      |     if ~strcmp(fltLambdaW_bkup,tmps)
      |       set_param(gcb,'fltLambdaW',tmps);
      |     end
      |   end
      |   if isnan(fltPropGainQ)
      |     if ~strcmp(fltPropGainQ_bkup,'0')
      |       set_param(gcb,'fltPropGainQ','0');
      |     end
      |   else
      |     tmps=num2str(fltPropGainQ);
      |     if ~strcmp(fltPropGainQ_bkup,tmps)
      |       set_param(gcb,'fltPropGainQ',tmps);
      |     end
      |   end
      |   if isnan(fltIntegGainQ)
      |     if ~strcmp(fltIntegGainQ_bkup,'0')
      |       set_param(gcb,'fltIntegGainQ','0');
      |     end
      |   else
      |     tmps=num2str(fltIntegGainQ);
      |     if ~strcmp(fltIntegGainQ_bkup,tmps)
      |       set_param(gcb,'fltIntegGainQ',tmps);
      |     end
      |   end
      |   if isnan(fltLowerLimitQ)
      |     if ~strcmp(fltLowerLimitQ_bkup,'0')
      |       set_param(gcb,'fltLowerLimitQ','0');
      |     end
      |   else
      |     tmps=num2str(fltLowerLimitQ);
      |     if ~strcmp(fltLowerLimitQ_bkup,tmps)
      |       set_param(gcb,'fltLowerLimitQ',tmps);
      |     end
      |   end
      |   if isnan(fltUpperLimitQ)
      |     if ~strcmp(fltUpperLimitQ_bkup,'0')
      |       set_param(gcb,'fltUpperLimitQ','0');
      |     end
      |   else
      |     tmps=num2str(fltUpperLimitQ);
      |     if ~strcmp(fltUpperLimitQ_bkup,tmps)
      |       set_param(gcb,'fltUpperLimitQ',tmps);
      |     end
      |   end
      |   if isnan(fltRampUp)
      |     if ~strcmp(fltRampUp_bkup,'0')
      |       set_param(gcb,'fltRampUp','0');
      |     end
      |   else
      |     tmps=num2str(fltRampUp);
      |     if ~strcmp(fltRampUp_bkup,tmps)
      |       set_param(gcb,'fltRampUp',tmps);
      |     end
      |   end
      |   if isnan(fltRampDown)
      |     if ~strcmp(fltRampDown_bkup,'0')
      |       set_param(gcb,'fltRampDown','0');
      |     end
      |   else
      |     tmps=num2str(fltRampDown);
      |     if ~strcmp(fltRampDown_bkup,tmps)
      |       set_param(gcb,'fltRampDown',tmps);
      |     end
      |   end
      | end
      mask Callback wksi:
      | autoCalcEn=get_param(gcb,'autoCalcEn');
      | if strcmp(autoCalcEn,'on')
      |   SampleTime=Simulink.data.evalinGlobal(bdroot,get_param(gcb,'SampleTime'));
      |   if (SampleTime==-1)
      |     SampleTime=str2double(get_param(gcb,'SampleTime_1'));
      |   end
      |   fltLambdaW_bkup=get_param(gcb,'fltLambdaW');
      |   fltPropGainQ_bkup=get_param(gcb,'fltPropGainQ');
      |   fltIntegGainQ_bkup=get_param(gcb,'fltIntegGainQ');
      |   fltLowerLimitQ_bkup=get_param(gcb,'fltLowerLimitQ');
      |   fltUpperLimitQ_bkup=get_param(gcb,'fltUpperLimitQ');
      |   fltRampUp_bkup=get_param(gcb,'fltRampUp');
      |   fltRampDown_bkup=get_param(gcb,'fltRampDown');
      |   wf0=Simulink.data.evalinGlobal(bdroot,get_param(gcb,'wf0'));
      |   wksi=Simulink.data.evalinGlobal(bdroot,get_param(gcb,'wksi'));
      |   J=Simulink.data.evalinGlobal(bdroot,get_param(gcb,'J'));
      |   Kt=Simulink.data.evalinGlobal(bdroot,get_param(gcb,'Kt'));
      |   lambdaW=Simulink.data.evalinGlobal(bdroot,get_param(gcb,'lambdaW'));
      |   ramprpm=Simulink.data.evalinGlobal(bdroot,get_param(gcb,'ramprpm'));
      |   mechspeed=Simulink.data.evalinGlobal(bdroot,get_param(gcb,'mechspeed'));
      |   polepairs=Simulink.data.evalinGlobal(bdroot,get_param(gcb,'polepairs'));
      |   if (wf0<=0)
      |     warning('Natural frequency f0 must be positive.');
      |   end
      |   if (wksi<=0)
      |     warning('Current loop attenuation must be positive.');
      |   end
      |   if (wksi>1)
      |     warning('Current loop attenuation must not exceed 1.');
      |   end
      |   if (J<=0)
      |     warning('Moment of inertia J must be positive.');
      |   end
      |   if (Kt<=0)
      |     warning('Torque constant Kt must be positive.');
      |   end
      |   if (lambdaW<0)
      |     warning('MA filter smoothing factor must be in the range 0..1.');
      |   end
      |   if (lambdaW>1)
      |     warning('MA filter smoothing factor must be in the range 0..1.');
      |   end
      |   if (mechspeed<=0)
      |     warning('Max. speed must be positive.');
      |   end
      |   if (polepairs<1)
      |     warning('Number of pole pairs must be a natural number (1, 2, 3, ...).');
      |   end
      |   if (round(polepairs)~=polepairs)
      |     warning('Number of pole pairs must be a natural number (1, 2, 3, ...).');
      |   end
      |   w0=6.283185307179586*wf0;
      |   pgain=2.0*wksi*w0*J/Kt;
      |   igain=w0*w0*J/Kt;
      |   wmax=polepairs*mechspeed*0.1047197551196598;
      |   fltPropGainQ=pgain;
      |   fltIntegGainQ=igain*SampleTime*0.5;
      |   fltLowerLimitQ=-wmax;
      |   fltUpperLimitQ=wmax;
      |   fltLambdaW=lambdaW;
      |   rampsc=polepairs*abs(ramprpm)*0.1047197551196598;
      |   fltRampUp=rampsc;
      |   fltRampDown=rampsc;
      |   if isnan(fltLambdaW)
      |     if ~strcmp(fltLambdaW_bkup,'0')
      |       set_param(gcb,'fltLambdaW','0');
      |     end
      |   else
      |     tmps=num2str(fltLambdaW);
      |     if ~strcmp(fltLambdaW_bkup,tmps)
      |       set_param(gcb,'fltLambdaW',tmps);
      |     end
      |   end
      |   if isnan(fltPropGainQ)
      |     if ~strcmp(fltPropGainQ_bkup,'0')
      |       set_param(gcb,'fltPropGainQ','0');
      |     end
      |   else
      |     tmps=num2str(fltPropGainQ);
      |     if ~strcmp(fltPropGainQ_bkup,tmps)
      |       set_param(gcb,'fltPropGainQ',tmps);
      |     end
      |   end
      |   if isnan(fltIntegGainQ)
      |     if ~strcmp(fltIntegGainQ_bkup,'0')
      |       set_param(gcb,'fltIntegGainQ','0');
      |     end
      |   else
      |     tmps=num2str(fltIntegGainQ);
      |     if ~strcmp(fltIntegGainQ_bkup,tmps)
      |       set_param(gcb,'fltIntegGainQ',tmps);
      |     end
      |   end
      |   if isnan(fltLowerLimitQ)
      |     if ~strcmp(fltLowerLimitQ_bkup,'0')
      |       set_param(gcb,'fltLowerLimitQ','0');
      |     end
      |   else
      |     tmps=num2str(fltLowerLimitQ);
      |     if ~strcmp(fltLowerLimitQ_bkup,tmps)
      |       set_param(gcb,'fltLowerLimitQ',tmps);
      |     end
      |   end
      |   if isnan(fltUpperLimitQ)
      |     if ~strcmp(fltUpperLimitQ_bkup,'0')
      |       set_param(gcb,'fltUpperLimitQ','0');
      |     end
      |   else
      |     tmps=num2str(fltUpperLimitQ);
      |     if ~strcmp(fltUpperLimitQ_bkup,tmps)
      |       set_param(gcb,'fltUpperLimitQ',tmps);
      |     end
      |   end
      |   if isnan(fltRampUp)
      |     if ~strcmp(fltRampUp_bkup,'0')
      |       set_param(gcb,'fltRampUp','0');
      |     end
      |   else
      |     tmps=num2str(fltRampUp);
      |     if ~strcmp(fltRampUp_bkup,tmps)
      |       set_param(gcb,'fltRampUp',tmps);
      |     end
      |   end
      |   if isnan(fltRampDown)
      |     if ~strcmp(fltRampDown_bkup,'0')
      |       set_param(gcb,'fltRampDown','0');
      |     end
      |   else
      |     tmps=num2str(fltRampDown);
      |     if ~strcmp(fltRampDown_bkup,tmps)
      |       set_param(gcb,'fltRampDown',tmps);
      |     end
      |   end
      | end
      mask Callback J:
      | autoCalcEn=get_param(gcb,'autoCalcEn');
      | if strcmp(autoCalcEn,'on')
      |   SampleTime=Simulink.data.evalinGlobal(bdroot,get_param(gcb,'SampleTime'));
      |   if (SampleTime==-1)
      |     SampleTime=str2double(get_param(gcb,'SampleTime_1'));
      |   end
      |   fltLambdaW_bkup=get_param(gcb,'fltLambdaW');
      |   fltPropGainQ_bkup=get_param(gcb,'fltPropGainQ');
      |   fltIntegGainQ_bkup=get_param(gcb,'fltIntegGainQ');
      |   fltLowerLimitQ_bkup=get_param(gcb,'fltLowerLimitQ');
      |   fltUpperLimitQ_bkup=get_param(gcb,'fltUpperLimitQ');
      |   fltRampUp_bkup=get_param(gcb,'fltRampUp');
      |   fltRampDown_bkup=get_param(gcb,'fltRampDown');
      |   wf0=Simulink.data.evalinGlobal(bdroot,get_param(gcb,'wf0'));
      |   wksi=Simulink.data.evalinGlobal(bdroot,get_param(gcb,'wksi'));
      |   J=Simulink.data.evalinGlobal(bdroot,get_param(gcb,'J'));
      |   Kt=Simulink.data.evalinGlobal(bdroot,get_param(gcb,'Kt'));
      |   lambdaW=Simulink.data.evalinGlobal(bdroot,get_param(gcb,'lambdaW'));
      |   ramprpm=Simulink.data.evalinGlobal(bdroot,get_param(gcb,'ramprpm'));
      |   mechspeed=Simulink.data.evalinGlobal(bdroot,get_param(gcb,'mechspeed'));
      |   polepairs=Simulink.data.evalinGlobal(bdroot,get_param(gcb,'polepairs'));
      |   if (wf0<=0)
      |     warning('Natural frequency f0 must be positive.');
      |   end
      |   if (wksi<=0)
      |     warning('Current loop attenuation must be positive.');
      |   end
      |   if (wksi>1)
      |     warning('Current loop attenuation must not exceed 1.');
      |   end
      |   if (J<=0)
      |     warning('Moment of inertia J must be positive.');
      |   end
      |   if (Kt<=0)
      |     warning('Torque constant Kt must be positive.');
      |   end
      |   if (lambdaW<0)
      |     warning('MA filter smoothing factor must be in the range 0..1.');
      |   end
      |   if (lambdaW>1)
      |     warning('MA filter smoothing factor must be in the range 0..1.');
      |   end
      |   if (mechspeed<=0)
      |     warning('Max. speed must be positive.');
      |   end
      |   if (polepairs<1)
      |     warning('Number of pole pairs must be a natural number (1, 2, 3, ...).');
      |   end
      |   if (round(polepairs)~=polepairs)
      |     warning('Number of pole pairs must be a natural number (1, 2, 3, ...).');
      |   end
      |   w0=6.283185307179586*wf0;
      |   pgain=2.0*wksi*w0*J/Kt;
      |   igain=w0*w0*J/Kt;
      |   wmax=polepairs*mechspeed*0.1047197551196598;
      |   fltPropGainQ=pgain;
      |   fltIntegGainQ=igain*SampleTime*0.5;
      |   fltLowerLimitQ=-wmax;
      |   fltUpperLimitQ=wmax;
      |   fltLambdaW=lambdaW;
      |   rampsc=polepairs*abs(ramprpm)*0.1047197551196598;
      |   fltRampUp=rampsc;
      |   fltRampDown=rampsc;
      |   if isnan(fltLambdaW)
      |     if ~strcmp(fltLambdaW_bkup,'0')
      |       set_param(gcb,'fltLambdaW','0');
      |     end
      |   else
      |     tmps=num2str(fltLambdaW);
      |     if ~strcmp(fltLambdaW_bkup,tmps)
      |       set_param(gcb,'fltLambdaW',tmps);
      |     end
      |   end
      |   if isnan(fltPropGainQ)
      |     if ~strcmp(fltPropGainQ_bkup,'0')
      |       set_param(gcb,'fltPropGainQ','0');
      |     end
      |   else
      |     tmps=num2str(fltPropGainQ);
      |     if ~strcmp(fltPropGainQ_bkup,tmps)
      |       set_param(gcb,'fltPropGainQ',tmps);
      |     end
      |   end
      |   if isnan(fltIntegGainQ)
      |     if ~strcmp(fltIntegGainQ_bkup,'0')
      |       set_param(gcb,'fltIntegGainQ','0');
      |     end
      |   else
      |     tmps=num2str(fltIntegGainQ);
      |     if ~strcmp(fltIntegGainQ_bkup,tmps)
      |       set_param(gcb,'fltIntegGainQ',tmps);
      |     end
      |   end
      |   if isnan(fltLowerLimitQ)
      |     if ~strcmp(fltLowerLimitQ_bkup,'0')
      |       set_param(gcb,'fltLowerLimitQ','0');
      |     end
      |   else
      |     tmps=num2str(fltLowerLimitQ);
      |     if ~strcmp(fltLowerLimitQ_bkup,tmps)
      |       set_param(gcb,'fltLowerLimitQ',tmps);
      |     end
      |   end
      |   if isnan(fltUpperLimitQ)
      |     if ~strcmp(fltUpperLimitQ_bkup,'0')
      |       set_param(gcb,'fltUpperLimitQ','0');
      |     end
      |   else
      |     tmps=num2str(fltUpperLimitQ);
      |     if ~strcmp(fltUpperLimitQ_bkup,tmps)
      |       set_param(gcb,'fltUpperLimitQ',tmps);
      |     end
      |   end
      |   if isnan(fltRampUp)
      |     if ~strcmp(fltRampUp_bkup,'0')
      |       set_param(gcb,'fltRampUp','0');
      |     end
      |   else
      |     tmps=num2str(fltRampUp);
      |     if ~strcmp(fltRampUp_bkup,tmps)
      |       set_param(gcb,'fltRampUp',tmps);
      |     end
      |   end
      |   if isnan(fltRampDown)
      |     if ~strcmp(fltRampDown_bkup,'0')
      |       set_param(gcb,'fltRampDown','0');
      |     end
      |   else
      |     tmps=num2str(fltRampDown);
      |     if ~strcmp(fltRampDown_bkup,tmps)
      |       set_param(gcb,'fltRampDown',tmps);
      |     end
      |   end
      | end
      mask Callback Kt:
      | autoCalcEn=get_param(gcb,'autoCalcEn');
      | if strcmp(autoCalcEn,'on')
      |   SampleTime=Simulink.data.evalinGlobal(bdroot,get_param(gcb,'SampleTime'));
      |   if (SampleTime==-1)
      |     SampleTime=str2double(get_param(gcb,'SampleTime_1'));
      |   end
      |   fltLambdaW_bkup=get_param(gcb,'fltLambdaW');
      |   fltPropGainQ_bkup=get_param(gcb,'fltPropGainQ');
      |   fltIntegGainQ_bkup=get_param(gcb,'fltIntegGainQ');
      |   fltLowerLimitQ_bkup=get_param(gcb,'fltLowerLimitQ');
      |   fltUpperLimitQ_bkup=get_param(gcb,'fltUpperLimitQ');
      |   fltRampUp_bkup=get_param(gcb,'fltRampUp');
      |   fltRampDown_bkup=get_param(gcb,'fltRampDown');
      |   wf0=Simulink.data.evalinGlobal(bdroot,get_param(gcb,'wf0'));
      |   wksi=Simulink.data.evalinGlobal(bdroot,get_param(gcb,'wksi'));
      |   J=Simulink.data.evalinGlobal(bdroot,get_param(gcb,'J'));
      |   Kt=Simulink.data.evalinGlobal(bdroot,get_param(gcb,'Kt'));
      |   lambdaW=Simulink.data.evalinGlobal(bdroot,get_param(gcb,'lambdaW'));
      |   ramprpm=Simulink.data.evalinGlobal(bdroot,get_param(gcb,'ramprpm'));
      |   mechspeed=Simulink.data.evalinGlobal(bdroot,get_param(gcb,'mechspeed'));
      |   polepairs=Simulink.data.evalinGlobal(bdroot,get_param(gcb,'polepairs'));
      |   if (wf0<=0)
      |     warning('Natural frequency f0 must be positive.');
      |   end
      |   if (wksi<=0)
      |     warning('Current loop attenuation must be positive.');
      |   end
      |   if (wksi>1)
      |     warning('Current loop attenuation must not exceed 1.');
      |   end
      |   if (J<=0)
      |     warning('Moment of inertia J must be positive.');
      |   end
      |   if (Kt<=0)
      |     warning('Torque constant Kt must be positive.');
      |   end
      |   if (lambdaW<0)
      |     warning('MA filter smoothing factor must be in the range 0..1.');
      |   end
      |   if (lambdaW>1)
      |     warning('MA filter smoothing factor must be in the range 0..1.');
      |   end
      |   if (mechspeed<=0)
      |     warning('Max. speed must be positive.');
      |   end
      |   if (polepairs<1)
      |     warning('Number of pole pairs must be a natural number (1, 2, 3, ...).');
      |   end
      |   if (round(polepairs)~=polepairs)
      |     warning('Number of pole pairs must be a natural number (1, 2, 3, ...).');
      |   end
      |   w0=6.283185307179586*wf0;
      |   pgain=2.0*wksi*w0*J/Kt;
      |   igain=w0*w0*J/Kt;
      |   wmax=polepairs*mechspeed*0.1047197551196598;
      |   fltPropGainQ=pgain;
      |   fltIntegGainQ=igain*SampleTime*0.5;
      |   fltLowerLimitQ=-wmax;
      |   fltUpperLimitQ=wmax;
      |   fltLambdaW=lambdaW;
      |   rampsc=polepairs*abs(ramprpm)*0.1047197551196598;
      |   fltRampUp=rampsc;
      |   fltRampDown=rampsc;
      |   if isnan(fltLambdaW)
      |     if ~strcmp(fltLambdaW_bkup,'0')
      |       set_param(gcb,'fltLambdaW','0');
      |     end
      |   else
      |     tmps=num2str(fltLambdaW);
      |     if ~strcmp(fltLambdaW_bkup,tmps)
      |       set_param(gcb,'fltLambdaW',tmps);
      |     end
      |   end
      |   if isnan(fltPropGainQ)
      |     if ~strcmp(fltPropGainQ_bkup,'0')
      |       set_param(gcb,'fltPropGainQ','0');
      |     end
      |   else
      |     tmps=num2str(fltPropGainQ);
      |     if ~strcmp(fltPropGainQ_bkup,tmps)
      |       set_param(gcb,'fltPropGainQ',tmps);
      |     end
      |   end
      |   if isnan(fltIntegGainQ)
      |     if ~strcmp(fltIntegGainQ_bkup,'0')
      |       set_param(gcb,'fltIntegGainQ','0');
      |     end
      |   else
      |     tmps=num2str(fltIntegGainQ);
      |     if ~strcmp(fltIntegGainQ_bkup,tmps)
      |       set_param(gcb,'fltIntegGainQ',tmps);
      |     end
      |   end
      |   if isnan(fltLowerLimitQ)
      |     if ~strcmp(fltLowerLimitQ_bkup,'0')
      |       set_param(gcb,'fltLowerLimitQ','0');
      |     end
      |   else
      |     tmps=num2str(fltLowerLimitQ);
      |     if ~strcmp(fltLowerLimitQ_bkup,tmps)
      |       set_param(gcb,'fltLowerLimitQ',tmps);
      |     end
      |   end
      |   if isnan(fltUpperLimitQ)
      |     if ~strcmp(fltUpperLimitQ_bkup,'0')
      |       set_param(gcb,'fltUpperLimitQ','0');
      |     end
      |   else
      |     tmps=num2str(fltUpperLimitQ);
      |     if ~strcmp(fltUpperLimitQ_bkup,tmps)
      |       set_param(gcb,'fltUpperLimitQ',tmps);
      |     end
      |   end
      |   if isnan(fltRampUp)
      |     if ~strcmp(fltRampUp_bkup,'0')
      |       set_param(gcb,'fltRampUp','0');
      |     end
      |   else
      |     tmps=num2str(fltRampUp);
      |     if ~strcmp(fltRampUp_bkup,tmps)
      |       set_param(gcb,'fltRampUp',tmps);
      |     end
      |   end
      |   if isnan(fltRampDown)
      |     if ~strcmp(fltRampDown_bkup,'0')
      |       set_param(gcb,'fltRampDown','0');
      |     end
      |   else
      |     tmps=num2str(fltRampDown);
      |     if ~strcmp(fltRampDown_bkup,tmps)
      |       set_param(gcb,'fltRampDown',tmps);
      |     end
      |   end
      | end
      mask Callback lambdaW:
      | autoCalcEn=get_param(gcb,'autoCalcEn');
      | if strcmp(autoCalcEn,'on')
      |   SampleTime=Simulink.data.evalinGlobal(bdroot,get_param(gcb,'SampleTime'));
      |   if (SampleTime==-1)
      |     SampleTime=str2double(get_param(gcb,'SampleTime_1'));
      |   end
      |   fltLambdaW_bkup=get_param(gcb,'fltLambdaW');
      |   fltPropGainQ_bkup=get_param(gcb,'fltPropGainQ');
      |   fltIntegGainQ_bkup=get_param(gcb,'fltIntegGainQ');
      |   fltLowerLimitQ_bkup=get_param(gcb,'fltLowerLimitQ');
      |   fltUpperLimitQ_bkup=get_param(gcb,'fltUpperLimitQ');
      |   fltRampUp_bkup=get_param(gcb,'fltRampUp');
      |   fltRampDown_bkup=get_param(gcb,'fltRampDown');
      |   wf0=Simulink.data.evalinGlobal(bdroot,get_param(gcb,'wf0'));
      |   wksi=Simulink.data.evalinGlobal(bdroot,get_param(gcb,'wksi'));
      |   J=Simulink.data.evalinGlobal(bdroot,get_param(gcb,'J'));
      |   Kt=Simulink.data.evalinGlobal(bdroot,get_param(gcb,'Kt'));
      |   lambdaW=Simulink.data.evalinGlobal(bdroot,get_param(gcb,'lambdaW'));
      |   ramprpm=Simulink.data.evalinGlobal(bdroot,get_param(gcb,'ramprpm'));
      |   mechspeed=Simulink.data.evalinGlobal(bdroot,get_param(gcb,'mechspeed'));
      |   polepairs=Simulink.data.evalinGlobal(bdroot,get_param(gcb,'polepairs'));
      |   if (wf0<=0)
      |     warning('Natural frequency f0 must be positive.');
      |   end
      |   if (wksi<=0)
      |     warning('Current loop attenuation must be positive.');
      |   end
      |   if (wksi>1)
      |     warning('Current loop attenuation must not exceed 1.');
      |   end
      |   if (J<=0)
      |     warning('Moment of inertia J must be positive.');
      |   end
      |   if (Kt<=0)
      |     warning('Torque constant Kt must be positive.');
      |   end
      |   if (lambdaW<0)
      |     warning('MA filter smoothing factor must be in the range 0..1.');
      |   end
      |   if (lambdaW>1)
      |     warning('MA filter smoothing factor must be in the range 0..1.');
      |   end
      |   if (mechspeed<=0)
      |     warning('Max. speed must be positive.');
      |   end
      |   if (polepairs<1)
      |     warning('Number of pole pairs must be a natural number (1, 2, 3, ...).');
      |   end
      |   if (round(polepairs)~=polepairs)
      |     warning('Number of pole pairs must be a natural number (1, 2, 3, ...).');
      |   end
      |   w0=6.283185307179586*wf0;
      |   pgain=2.0*wksi*w0*J/Kt;
      |   igain=w0*w0*J/Kt;
      |   wmax=polepairs*mechspeed*0.1047197551196598;
      |   fltPropGainQ=pgain;
      |   fltIntegGainQ=igain*SampleTime*0.5;
      |   fltLowerLimitQ=-wmax;
      |   fltUpperLimitQ=wmax;
      |   fltLambdaW=lambdaW;
      |   rampsc=polepairs*abs(ramprpm)*0.1047197551196598;
      |   fltRampUp=rampsc;
      |   fltRampDown=rampsc;
      |   if isnan(fltLambdaW)
      |     if ~strcmp(fltLambdaW_bkup,'0')
      |       set_param(gcb,'fltLambdaW','0');
      |     end
      |   else
      |     tmps=num2str(fltLambdaW);
      |     if ~strcmp(fltLambdaW_bkup,tmps)
      |       set_param(gcb,'fltLambdaW',tmps);
      |     end
      |   end
      |   if isnan(fltPropGainQ)
      |     if ~strcmp(fltPropGainQ_bkup,'0')
      |       set_param(gcb,'fltPropGainQ','0');
      |     end
      |   else
      |     tmps=num2str(fltPropGainQ);
      |     if ~strcmp(fltPropGainQ_bkup,tmps)
      |       set_param(gcb,'fltPropGainQ',tmps);
      |     end
      |   end
      |   if isnan(fltIntegGainQ)
      |     if ~strcmp(fltIntegGainQ_bkup,'0')
      |       set_param(gcb,'fltIntegGainQ','0');
      |     end
      |   else
      |     tmps=num2str(fltIntegGainQ);
      |     if ~strcmp(fltIntegGainQ_bkup,tmps)
      |       set_param(gcb,'fltIntegGainQ',tmps);
      |     end
      |   end
      |   if isnan(fltLowerLimitQ)
      |     if ~strcmp(fltLowerLimitQ_bkup,'0')
      |       set_param(gcb,'fltLowerLimitQ','0');
      |     end
      |   else
      |     tmps=num2str(fltLowerLimitQ);
      |     if ~strcmp(fltLowerLimitQ_bkup,tmps)
      |       set_param(gcb,'fltLowerLimitQ',tmps);
      |     end
      |   end
      |   if isnan(fltUpperLimitQ)
      |     if ~strcmp(fltUpperLimitQ_bkup,'0')
      |       set_param(gcb,'fltUpperLimitQ','0');
      |     end
      |   else
      |     tmps=num2str(fltUpperLimitQ);
      |     if ~strcmp(fltUpperLimitQ_bkup,tmps)
      |       set_param(gcb,'fltUpperLimitQ',tmps);
      |     end
      |   end
      |   if isnan(fltRampUp)
      |     if ~strcmp(fltRampUp_bkup,'0')
      |       set_param(gcb,'fltRampUp','0');
      |     end
      |   else
      |     tmps=num2str(fltRampUp);
      |     if ~strcmp(fltRampUp_bkup,tmps)
      |       set_param(gcb,'fltRampUp',tmps);
      |     end
      |   end
      |   if isnan(fltRampDown)
      |     if ~strcmp(fltRampDown_bkup,'0')
      |       set_param(gcb,'fltRampDown','0');
      |     end
      |   else
      |     tmps=num2str(fltRampDown);
      |     if ~strcmp(fltRampDown_bkup,tmps)
      |       set_param(gcb,'fltRampDown',tmps);
      |     end
      |   end
      | end
      mask Callback ramprpm:
      | autoCalcEn=get_param(gcb,'autoCalcEn');
      | if strcmp(autoCalcEn,'on')
      |   SampleTime=Simulink.data.evalinGlobal(bdroot,get_param(gcb,'SampleTime'));
      |   if (SampleTime==-1)
      |     SampleTime=str2double(get_param(gcb,'SampleTime_1'));
      |   end
      |   fltLambdaW_bkup=get_param(gcb,'fltLambdaW');
      |   fltPropGainQ_bkup=get_param(gcb,'fltPropGainQ');
      |   fltIntegGainQ_bkup=get_param(gcb,'fltIntegGainQ');
      |   fltLowerLimitQ_bkup=get_param(gcb,'fltLowerLimitQ');
      |   fltUpperLimitQ_bkup=get_param(gcb,'fltUpperLimitQ');
      |   fltRampUp_bkup=get_param(gcb,'fltRampUp');
      |   fltRampDown_bkup=get_param(gcb,'fltRampDown');
      |   wf0=Simulink.data.evalinGlobal(bdroot,get_param(gcb,'wf0'));
      |   wksi=Simulink.data.evalinGlobal(bdroot,get_param(gcb,'wksi'));
      |   J=Simulink.data.evalinGlobal(bdroot,get_param(gcb,'J'));
      |   Kt=Simulink.data.evalinGlobal(bdroot,get_param(gcb,'Kt'));
      |   lambdaW=Simulink.data.evalinGlobal(bdroot,get_param(gcb,'lambdaW'));
      |   ramprpm=Simulink.data.evalinGlobal(bdroot,get_param(gcb,'ramprpm'));
      |   mechspeed=Simulink.data.evalinGlobal(bdroot,get_param(gcb,'mechspeed'));
      |   polepairs=Simulink.data.evalinGlobal(bdroot,get_param(gcb,'polepairs'));
      |   if (wf0<=0)
      |     warning('Natural frequency f0 must be positive.');
      |   end
      |   if (wksi<=0)
      |     warning('Current loop attenuation must be positive.');
      |   end
      |   if (wksi>1)
      |     warning('Current loop attenuation must not exceed 1.');
      |   end
      |   if (J<=0)
      |     warning('Moment of inertia J must be positive.');
      |   end
      |   if (Kt<=0)
      |     warning('Torque constant Kt must be positive.');
      |   end
      |   if (lambdaW<0)
      |     warning('MA filter smoothing factor must be in the range 0..1.');
      |   end
      |   if (lambdaW>1)
      |     warning('MA filter smoothing factor must be in the range 0..1.');
      |   end
      |   if (mechspeed<=0)
      |     warning('Max. speed must be positive.');
      |   end
      |   if (polepairs<1)
      |     warning('Number of pole pairs must be a natural number (1, 2, 3, ...).');
      |   end
      |   if (round(polepairs)~=polepairs)
      |     warning('Number of pole pairs must be a natural number (1, 2, 3, ...).');
      |   end
      |   w0=6.283185307179586*wf0;
      |   pgain=2.0*wksi*w0*J/Kt;
      |   igain=w0*w0*J/Kt;
      |   wmax=polepairs*mechspeed*0.1047197551196598;
      |   fltPropGainQ=pgain;
      |   fltIntegGainQ=igain*SampleTime*0.5;
      |   fltLowerLimitQ=-wmax;
      |   fltUpperLimitQ=wmax;
      |   fltLambdaW=lambdaW;
      |   rampsc=polepairs*abs(ramprpm)*0.1047197551196598;
      |   fltRampUp=rampsc;
      |   fltRampDown=rampsc;
      |   if isnan(fltLambdaW)
      |     if ~strcmp(fltLambdaW_bkup,'0')
      |       set_param(gcb,'fltLambdaW','0');
      |     end
      |   else
      |     tmps=num2str(fltLambdaW);
      |     if ~strcmp(fltLambdaW_bkup,tmps)
      |       set_param(gcb,'fltLambdaW',tmps);
      |     end
      |   end
      |   if isnan(fltPropGainQ)
      |     if ~strcmp(fltPropGainQ_bkup,'0')
      |       set_param(gcb,'fltPropGainQ','0');
      |     end
      |   else
      |     tmps=num2str(fltPropGainQ);
      |     if ~strcmp(fltPropGainQ_bkup,tmps)
      |       set_param(gcb,'fltPropGainQ',tmps);
      |     end
      |   end
      |   if isnan(fltIntegGainQ)
      |     if ~strcmp(fltIntegGainQ_bkup,'0')
      |       set_param(gcb,'fltIntegGainQ','0');
      |     end
      |   else
      |     tmps=num2str(fltIntegGainQ);
      |     if ~strcmp(fltIntegGainQ_bkup,tmps)
      |       set_param(gcb,'fltIntegGainQ',tmps);
      |     end
      |   end
      |   if isnan(fltLowerLimitQ)
      |     if ~strcmp(fltLowerLimitQ_bkup,'0')
      |       set_param(gcb,'fltLowerLimitQ','0');
      |     end
      |   else
      |     tmps=num2str(fltLowerLimitQ);
      |     if ~strcmp(fltLowerLimitQ_bkup,tmps)
      |       set_param(gcb,'fltLowerLimitQ',tmps);
      |     end
      |   end
      |   if isnan(fltUpperLimitQ)
      |     if ~strcmp(fltUpperLimitQ_bkup,'0')
      |       set_param(gcb,'fltUpperLimitQ','0');
      |     end
      |   else
      |     tmps=num2str(fltUpperLimitQ);
      |     if ~strcmp(fltUpperLimitQ_bkup,tmps)
      |       set_param(gcb,'fltUpperLimitQ',tmps);
      |     end
      |   end
      |   if isnan(fltRampUp)
      |     if ~strcmp(fltRampUp_bkup,'0')
      |       set_param(gcb,'fltRampUp','0');
      |     end
      |   else
      |     tmps=num2str(fltRampUp);
      |     if ~strcmp(fltRampUp_bkup,tmps)
      |       set_param(gcb,'fltRampUp',tmps);
      |     end
      |   end
      |   if isnan(fltRampDown)
      |     if ~strcmp(fltRampDown_bkup,'0')
      |       set_param(gcb,'fltRampDown','0');
      |     end
      |   else
      |     tmps=num2str(fltRampDown);
      |     if ~strcmp(fltRampDown_bkup,tmps)
      |       set_param(gcb,'fltRampDown',tmps);
      |     end
      |   end
      | end
      mask Callback mechspeed:
      | autoCalcEn=get_param(gcb,'autoCalcEn');
      | if strcmp(autoCalcEn,'on')
      |   SampleTime=Simulink.data.evalinGlobal(bdroot,get_param(gcb,'SampleTime'));
      |   if (SampleTime==-1)
      |     SampleTime=str2double(get_param(gcb,'SampleTime_1'));
      |   end
      |   fltLambdaW_bkup=get_param(gcb,'fltLambdaW');
      |   fltPropGainQ_bkup=get_param(gcb,'fltPropGainQ');
      |   fltIntegGainQ_bkup=get_param(gcb,'fltIntegGainQ');
      |   fltLowerLimitQ_bkup=get_param(gcb,'fltLowerLimitQ');
      |   fltUpperLimitQ_bkup=get_param(gcb,'fltUpperLimitQ');
      |   fltRampUp_bkup=get_param(gcb,'fltRampUp');
      |   fltRampDown_bkup=get_param(gcb,'fltRampDown');
      |   wf0=Simulink.data.evalinGlobal(bdroot,get_param(gcb,'wf0'));
      |   wksi=Simulink.data.evalinGlobal(bdroot,get_param(gcb,'wksi'));
      |   J=Simulink.data.evalinGlobal(bdroot,get_param(gcb,'J'));
      |   Kt=Simulink.data.evalinGlobal(bdroot,get_param(gcb,'Kt'));
      |   lambdaW=Simulink.data.evalinGlobal(bdroot,get_param(gcb,'lambdaW'));
      |   ramprpm=Simulink.data.evalinGlobal(bdroot,get_param(gcb,'ramprpm'));
      |   mechspeed=Simulink.data.evalinGlobal(bdroot,get_param(gcb,'mechspeed'));
      |   polepairs=Simulink.data.evalinGlobal(bdroot,get_param(gcb,'polepairs'));
      |   if (wf0<=0)
      |     warning('Natural frequency f0 must be positive.');
      |   end
      |   if (wksi<=0)
      |     warning('Current loop attenuation must be positive.');
      |   end
      |   if (wksi>1)
      |     warning('Current loop attenuation must not exceed 1.');
      |   end
      |   if (J<=0)
      |     warning('Moment of inertia J must be positive.');
      |   end
      |   if (Kt<=0)
      |     warning('Torque constant Kt must be positive.');
      |   end
      |   if (lambdaW<0)
      |     warning('MA filter smoothing factor must be in the range 0..1.');
      |   end
      |   if (lambdaW>1)
      |     warning('MA filter smoothing factor must be in the range 0..1.');
      |   end
      |   if (mechspeed<=0)
      |     warning('Max. speed must be positive.');
      |   end
      |   if (polepairs<1)
      |     warning('Number of pole pairs must be a natural number (1, 2, 3, ...).');
      |   end
      |   if (round(polepairs)~=polepairs)
      |     warning('Number of pole pairs must be a natural number (1, 2, 3, ...).');
      |   end
      |   w0=6.283185307179586*wf0;
      |   pgain=2.0*wksi*w0*J/Kt;
      |   igain=w0*w0*J/Kt;
      |   wmax=polepairs*mechspeed*0.1047197551196598;
      |   fltPropGainQ=pgain;
      |   fltIntegGainQ=igain*SampleTime*0.5;
      |   fltLowerLimitQ=-wmax;
      |   fltUpperLimitQ=wmax;
      |   fltLambdaW=lambdaW;
      |   rampsc=polepairs*abs(ramprpm)*0.1047197551196598;
      |   fltRampUp=rampsc;
      |   fltRampDown=rampsc;
      |   if isnan(fltLambdaW)
      |     if ~strcmp(fltLambdaW_bkup,'0')
      |       set_param(gcb,'fltLambdaW','0');
      |     end
      |   else
      |     tmps=num2str(fltLambdaW);
      |     if ~strcmp(fltLambdaW_bkup,tmps)
      |       set_param(gcb,'fltLambdaW',tmps);
      |     end
      |   end
      |   if isnan(fltPropGainQ)
      |     if ~strcmp(fltPropGainQ_bkup,'0')
      |       set_param(gcb,'fltPropGainQ','0');
      |     end
      |   else
      |     tmps=num2str(fltPropGainQ);
      |     if ~strcmp(fltPropGainQ_bkup,tmps)
      |       set_param(gcb,'fltPropGainQ',tmps);
      |     end
      |   end
      |   if isnan(fltIntegGainQ)
      |     if ~strcmp(fltIntegGainQ_bkup,'0')
      |       set_param(gcb,'fltIntegGainQ','0');
      |     end
      |   else
      |     tmps=num2str(fltIntegGainQ);
      |     if ~strcmp(fltIntegGainQ_bkup,tmps)
      |       set_param(gcb,'fltIntegGainQ',tmps);
      |     end
      |   end
      |   if isnan(fltLowerLimitQ)
      |     if ~strcmp(fltLowerLimitQ_bkup,'0')
      |       set_param(gcb,'fltLowerLimitQ','0');
      |     end
      |   else
      |     tmps=num2str(fltLowerLimitQ);
      |     if ~strcmp(fltLowerLimitQ_bkup,tmps)
      |       set_param(gcb,'fltLowerLimitQ',tmps);
      |     end
      |   end
      |   if isnan(fltUpperLimitQ)
      |     if ~strcmp(fltUpperLimitQ_bkup,'0')
      |       set_param(gcb,'fltUpperLimitQ','0');
      |     end
      |   else
      |     tmps=num2str(fltUpperLimitQ);
      |     if ~strcmp(fltUpperLimitQ_bkup,tmps)
      |       set_param(gcb,'fltUpperLimitQ',tmps);
      |     end
      |   end
      |   if isnan(fltRampUp)
      |     if ~strcmp(fltRampUp_bkup,'0')
      |       set_param(gcb,'fltRampUp','0');
      |     end
      |   else
      |     tmps=num2str(fltRampUp);
      |     if ~strcmp(fltRampUp_bkup,tmps)
      |       set_param(gcb,'fltRampUp',tmps);
      |     end
      |   end
      |   if isnan(fltRampDown)
      |     if ~strcmp(fltRampDown_bkup,'0')
      |       set_param(gcb,'fltRampDown','0');
      |     end
      |   else
      |     tmps=num2str(fltRampDown);
      |     if ~strcmp(fltRampDown_bkup,tmps)
      |       set_param(gcb,'fltRampDown',tmps);
      |     end
      |   end
      | end
      mask Callback polepairs:
      | autoCalcEn=get_param(gcb,'autoCalcEn');
      | if strcmp(autoCalcEn,'on')
      |   SampleTime=Simulink.data.evalinGlobal(bdroot,get_param(gcb,'SampleTime'));
      |   if (SampleTime==-1)
      |     SampleTime=str2double(get_param(gcb,'SampleTime_1'));
      |   end
      |   fltLambdaW_bkup=get_param(gcb,'fltLambdaW');
      |   fltPropGainQ_bkup=get_param(gcb,'fltPropGainQ');
      |   fltIntegGainQ_bkup=get_param(gcb,'fltIntegGainQ');
      |   fltLowerLimitQ_bkup=get_param(gcb,'fltLowerLimitQ');
      |   fltUpperLimitQ_bkup=get_param(gcb,'fltUpperLimitQ');
      |   fltRampUp_bkup=get_param(gcb,'fltRampUp');
      |   fltRampDown_bkup=get_param(gcb,'fltRampDown');
      |   wf0=Simulink.data.evalinGlobal(bdroot,get_param(gcb,'wf0'));
      |   wksi=Simulink.data.evalinGlobal(bdroot,get_param(gcb,'wksi'));
      |   J=Simulink.data.evalinGlobal(bdroot,get_param(gcb,'J'));
      |   Kt=Simulink.data.evalinGlobal(bdroot,get_param(gcb,'Kt'));
      |   lambdaW=Simulink.data.evalinGlobal(bdroot,get_param(gcb,'lambdaW'));
      |   ramprpm=Simulink.data.evalinGlobal(bdroot,get_param(gcb,'ramprpm'));
      |   mechspeed=Simulink.data.evalinGlobal(bdroot,get_param(gcb,'mechspeed'));
      |   polepairs=Simulink.data.evalinGlobal(bdroot,get_param(gcb,'polepairs'));
      |   if (wf0<=0)
      |     warning('Natural frequency f0 must be positive.');
      |   end
      |   if (wksi<=0)
      |     warning('Current loop attenuation must be positive.');
      |   end
      |   if (wksi>1)
      |     warning('Current loop attenuation must not exceed 1.');
      |   end
      |   if (J<=0)
      |     warning('Moment of inertia J must be positive.');
      |   end
      |   if (Kt<=0)
      |     warning('Torque constant Kt must be positive.');
      |   end
      |   if (lambdaW<0)
      |     warning('MA filter smoothing factor must be in the range 0..1.');
      |   end
      |   if (lambdaW>1)
      |     warning('MA filter smoothing factor must be in the range 0..1.');
      |   end
      |   if (mechspeed<=0)
      |     warning('Max. speed must be positive.');
      |   end
      |   if (polepairs<1)
      |     warning('Number of pole pairs must be a natural number (1, 2, 3, ...).');
      |   end
      |   if (round(polepairs)~=polepairs)
      |     warning('Number of pole pairs must be a natural number (1, 2, 3, ...).');
      |   end
      |   w0=6.283185307179586*wf0;
      |   pgain=2.0*wksi*w0*J/Kt;
      |   igain=w0*w0*J/Kt;
      |   wmax=polepairs*mechspeed*0.1047197551196598;
      |   fltPropGainQ=pgain;
      |   fltIntegGainQ=igain*SampleTime*0.5;
      |   fltLowerLimitQ=-wmax;
      |   fltUpperLimitQ=wmax;
      |   fltLambdaW=lambdaW;
      |   rampsc=polepairs*abs(ramprpm)*0.1047197551196598;
      |   fltRampUp=rampsc;
      |   fltRampDown=rampsc;
      |   if isnan(fltLambdaW)
      |     if ~strcmp(fltLambdaW_bkup,'0')
      |       set_param(gcb,'fltLambdaW','0');
      |     end
      |   else
      |     tmps=num2str(fltLambdaW);
      |     if ~strcmp(fltLambdaW_bkup,tmps)
      |       set_param(gcb,'fltLambdaW',tmps);
      |     end
      |   end
      |   if isnan(fltPropGainQ)
      |     if ~strcmp(fltPropGainQ_bkup,'0')
      |       set_param(gcb,'fltPropGainQ','0');
      |     end
      |   else
      |     tmps=num2str(fltPropGainQ);
      |     if ~strcmp(fltPropGainQ_bkup,tmps)
      |       set_param(gcb,'fltPropGainQ',tmps);
      |     end
      |   end
      |   if isnan(fltIntegGainQ)
      |     if ~strcmp(fltIntegGainQ_bkup,'0')
      |       set_param(gcb,'fltIntegGainQ','0');
      |     end
      |   else
      |     tmps=num2str(fltIntegGainQ);
      |     if ~strcmp(fltIntegGainQ_bkup,tmps)
      |       set_param(gcb,'fltIntegGainQ',tmps);
      |     end
      |   end
      |   if isnan(fltLowerLimitQ)
      |     if ~strcmp(fltLowerLimitQ_bkup,'0')
      |       set_param(gcb,'fltLowerLimitQ','0');
      |     end
      |   else
      |     tmps=num2str(fltLowerLimitQ);
      |     if ~strcmp(fltLowerLimitQ_bkup,tmps)
      |       set_param(gcb,'fltLowerLimitQ',tmps);
      |     end
      |   end
      |   if isnan(fltUpperLimitQ)
      |     if ~strcmp(fltUpperLimitQ_bkup,'0')
      |       set_param(gcb,'fltUpperLimitQ','0');
      |     end
      |   else
      |     tmps=num2str(fltUpperLimitQ);
      |     if ~strcmp(fltUpperLimitQ_bkup,tmps)
      |       set_param(gcb,'fltUpperLimitQ',tmps);
      |     end
      |   end
      |   if isnan(fltRampUp)
      |     if ~strcmp(fltRampUp_bkup,'0')
      |       set_param(gcb,'fltRampUp','0');
      |     end
      |   else
      |     tmps=num2str(fltRampUp);
      |     if ~strcmp(fltRampUp_bkup,tmps)
      |       set_param(gcb,'fltRampUp',tmps);
      |     end
      |   end
      |   if isnan(fltRampDown)
      |     if ~strcmp(fltRampDown_bkup,'0')
      |       set_param(gcb,'fltRampDown','0');
      |     end
      |   else
      |     tmps=num2str(fltRampDown);
      |     if ~strcmp(fltRampDown_bkup,tmps)
      |       set_param(gcb,'fltRampDown',tmps);
      |     end
      |   end
      | end
      mask Callback autoCalcEn:
      | maskStr=get_param(gcb,'showStates');
      | if strcmp(maskStr,'Hide (faster execution)')
      |   p=Simulink.Mask.get(gcb);
      |   autoCalcEn=get_param(gcb,'autoCalcEn');
      |   hintText=p.getDialogControl('timeHint');
      |   if strcmp(autoCalcEn,'on')
      |     param=p.getParameter('polepairs');
      |     if strcmp(param.Enabled,'off')
      |       SampleTime=Simulink.data.evalinGlobal(bdroot,get_param(gcb,'SampleTime'));
      |       if SampleTime==-1
      |         SampleTime=str2double(get_param(gcb,'SampleTime_1'));
      |         if isnan(SampleTime)
      |           hintText.Prompt=['Note: Implementation parameters cannot be calculated yet because the block''s inherited sample time is unknown. Simulink will update the sample time when you run the simulation.'];
      |         else
      |           hintText.Prompt=['Caution: Implementation parameters depend on inherited sample time. Make sure that the sample time of the block''s inputs corresponds to the sampling period in the target application.'];
      |         end
      |       else
      |         hintText.Prompt='Caution: Implementation parameters depend on the sample time. Make sure that the simulation time step corresponds to the sampling period in the target application.';
      |       end
      |       p=Simulink.Mask.get(gcb);
      |       param=p.getParameter('wf0');
      |       param.set('Enabled','on');
      |       param=p.getParameter('wksi');
      |       param.set('Enabled','on');
      |       param=p.getParameter('J');
      |       param.set('Enabled','on');
      |       param=p.getParameter('Kt');
      |       param.set('Enabled','on');
      |       param=p.getParameter('lambdaW');
      |       param.set('Enabled','on');
      |       param=p.getParameter('ramprpm');
      |       param.set('Enabled','on');
      |       param=p.getParameter('mechspeed');
      |       param.set('Enabled','on');
      |       param=p.getParameter('polepairs');
      |       param.set('Enabled','on');
      |     else
      |       SampleTime=Simulink.data.evalinGlobal(bdroot,get_param(gcb,'SampleTime'));
      |       if SampleTime==-1
      |         SampleTime=str2double(get_param(gcb,'SampleTime_1'));
      |       end
      |     end
      |     fltLambdaW_bkup=get_param(gcb,'fltLambdaW');
      |     fltPropGainQ_bkup=get_param(gcb,'fltPropGainQ');
      |     fltIntegGainQ_bkup=get_param(gcb,'fltIntegGainQ');
      |     fltLowerLimitQ_bkup=get_param(gcb,'fltLowerLimitQ');
      |     fltUpperLimitQ_bkup=get_param(gcb,'fltUpperLimitQ');
      |     fltRampUp_bkup=get_param(gcb,'fltRampUp');
      |     fltRampDown_bkup=get_param(gcb,'fltRampDown');
      |     wf0=Simulink.data.evalinGlobal(bdroot,get_param(gcb,'wf0'));
      |     wksi=Simulink.data.evalinGlobal(bdroot,get_param(gcb,'wksi'));
      |     J=Simulink.data.evalinGlobal(bdroot,get_param(gcb,'J'));
      |     Kt=Simulink.data.evalinGlobal(bdroot,get_param(gcb,'Kt'));
      |     lambdaW=Simulink.data.evalinGlobal(bdroot,get_param(gcb,'lambdaW'));
      |     ramprpm=Simulink.data.evalinGlobal(bdroot,get_param(gcb,'ramprpm'));
      |     mechspeed=Simulink.data.evalinGlobal(bdroot,get_param(gcb,'mechspeed'));
      |     polepairs=Simulink.data.evalinGlobal(bdroot,get_param(gcb,'polepairs'));
      |     if (wf0<=0)
      |       warning('Natural frequency f0 must be positive.');
      |     end
      |     if (wksi<=0)
      |       warning('Current loop attenuation must be positive.');
      |     end
      |     if (wksi>1)
      |       warning('Current loop attenuation must not exceed 1.');
      |     end
      |     if (J<=0)
      |       warning('Moment of inertia J must be positive.');
      |     end
      |     if (Kt<=0)
      |       warning('Torque constant Kt must be positive.');
      |     end
      |     if (lambdaW<0)
      |       warning('MA filter smoothing factor must be in the range 0..1.');
      |     end
      |     if (lambdaW>1)
      |       warning('MA filter smoothing factor must be in the range 0..1.');
      |     end
      |     if (mechspeed<=0)
      |       warning('Max. speed must be positive.');
      |     end
      |     if (polepairs<1)
      |       warning('Number of pole pairs must be a natural number (1, 2, 3, ...).');
      |     end
      |     if (round(polepairs)~=polepairs)
      |       warning('Number of pole pairs must be a natural number (1, 2, 3, ...).');
      |     end
      |     w0=6.283185307179586*wf0;
      |     pgain=2.0*wksi*w0*J/Kt;
      |     igain=w0*w0*J/Kt;
      |     wmax=polepairs*mechspeed*0.1047197551196598;
      |     fltPropGainQ=pgain;
      |     fltIntegGainQ=igain*SampleTime*0.5;
      |     fltLowerLimitQ=-wmax;
      |     fltUpperLimitQ=wmax;
      |     fltLambdaW=lambdaW;
      |     rampsc=polepairs*abs(ramprpm)*0.1047197551196598;
      |     fltRampUp=rampsc;
      |     fltRampDown=rampsc;
      |     if isnan(fltLambdaW)
      |       if ~strcmp(fltLambdaW_bkup,'0')
      |         set_param(gcb,'fltLambdaW','0');
      |       end
      |     else
      |       tmps=num2str(fltLambdaW);
      |       if ~strcmp(fltLambdaW_bkup,tmps)
      |         set_param(gcb,'fltLambdaW',tmps);
      |       end
      |     end
      |     if isnan(fltPropGainQ)
      |       if ~strcmp(fltPropGainQ_bkup,'0')
      |         set_param(gcb,'fltPropGainQ','0');
      |       end
      |     else
      |       tmps=num2str(fltPropGainQ);
      |       if ~strcmp(fltPropGainQ_bkup,tmps)
      |         set_param(gcb,'fltPropGainQ',tmps);
      |       end
      |     end
      |     if isnan(fltIntegGainQ)
      |       if ~strcmp(fltIntegGainQ_bkup,'0')
      |         set_param(gcb,'fltIntegGainQ','0');
      |       end
      |     else
      |       tmps=num2str(fltIntegGainQ);
      |       if ~strcmp(fltIntegGainQ_bkup,tmps)
      |         set_param(gcb,'fltIntegGainQ',tmps);
      |       end
      |     end
      |     if isnan(fltLowerLimitQ)
      |       if ~strcmp(fltLowerLimitQ_bkup,'0')
      |         set_param(gcb,'fltLowerLimitQ','0');
      |       end
      |     else
      |       tmps=num2str(fltLowerLimitQ);
      |       if ~strcmp(fltLowerLimitQ_bkup,tmps)
      |         set_param(gcb,'fltLowerLimitQ',tmps);
      |       end
      |     end
      |     if isnan(fltUpperLimitQ)
      |       if ~strcmp(fltUpperLimitQ_bkup,'0')
      |         set_param(gcb,'fltUpperLimitQ','0');
      |       end
      |     else
      |       tmps=num2str(fltUpperLimitQ);
      |       if ~strcmp(fltUpperLimitQ_bkup,tmps)
      |         set_param(gcb,'fltUpperLimitQ',tmps);
      |       end
      |     end
      |     if isnan(fltRampUp)
      |       if ~strcmp(fltRampUp_bkup,'0')
      |         set_param(gcb,'fltRampUp','0');
      |       end
      |     else
      |       tmps=num2str(fltRampUp);
      |       if ~strcmp(fltRampUp_bkup,tmps)
      |         set_param(gcb,'fltRampUp',tmps);
      |       end
      |     end
      |     if isnan(fltRampDown)
      |       if ~strcmp(fltRampDown_bkup,'0')
      |         set_param(gcb,'fltRampDown','0');
      |       end
      |     else
      |       tmps=num2str(fltRampDown);
      |       if ~strcmp(fltRampDown_bkup,tmps)
      |         set_param(gcb,'fltRampDown',tmps);
      |       end
      |     end
      |   else
      |     param=p.getParameter('polepairs');
      |     if strcmp(param.Enabled,'on')
      |       hintText.Prompt='Caution: Implementation parameters are fixed.';
      |       p=Simulink.Mask.get(gcb);
      |       param=p.getParameter('wf0');
      |       param.set('Enabled','off');
      |       param=p.getParameter('wksi');
      |       param.set('Enabled','off');
      |       param=p.getParameter('J');
      |       param.set('Enabled','off');
      |       param=p.getParameter('Kt');
      |       param.set('Enabled','off');
      |       param=p.getParameter('lambdaW');
      |       param.set('Enabled','off');
      |       param=p.getParameter('ramprpm');
      |       param.set('Enabled','off');
      |       param=p.getParameter('mechspeed');
      |       param.set('Enabled','off');
      |       param=p.getParameter('polepairs');
      |       param.set('Enabled','off');
      |     end
      |   end
      | end
      mask DialogControl CompBut Prompt: Recalculate sample times
      mask DialogControl CompBut Tooltip: Simulink updates the sample times of all blocks when the simulation is run. This button will update the sample times now.
      mask DialogControl CompBut Callback:
      | btn=questdlg('This will apply all changes in all open dialog boxes and update the schematic. Do you want to proceed?','Apply all changes','Continue','Cancel','Continue');
      | if strcmp(btn,'Continue')
      |   dlgs=DAStudio.ToolRoot.getOpenDialogs;
      |   for i=1:length(dlgs)
      |     dlgs(i).apply;
      |   end
      |   try
      |     SampleTime_1=str2double(get_param(gcb,'SampleTime_1'));
      |     ts=Simulink.Block.getSampleTimes(gcb);
      |     ts=ts(1).Value(1);
      |     if (SampleTime_1 ~= ts)
      |       SampleTime_1=ts;
      |       set_param(gcb,'SampleTime_1',num2str(ts));
      |       autoCalcEn=get_param(gcb,'autoCalcEn');
      |       if strcmp(autoCalcEn,'on')
      |         SampleTime=Simulink.data.evalinGlobal(bdroot,get_param(gcb,'SampleTime'));
      |         p=Simulink.Mask.get(gcb);
      |         hintText=p.getDialogControl('timeHint');
      |         if SampleTime==-1
      |           SampleTime=SampleTime_1;
      |           hintText.Prompt='Caution: Implementation parameters depend on inherited sample time. Make sure that the sample time of the block''s inputs corresponds to the sampling period in the target application.';
      |         else
      |           hintText.Prompt='Caution: Implementation parameters depend on the sample time. Make sure that the simulation time step corresponds to the sampling period in the target application.';
      |         end
      |         fltLambdaW_bkup=get_param(gcb,'fltLambdaW');
      |         fltPropGainQ_bkup=get_param(gcb,'fltPropGainQ');
      |         fltIntegGainQ_bkup=get_param(gcb,'fltIntegGainQ');
      |         fltLowerLimitQ_bkup=get_param(gcb,'fltLowerLimitQ');
      |         fltUpperLimitQ_bkup=get_param(gcb,'fltUpperLimitQ');
      |         fltRampUp_bkup=get_param(gcb,'fltRampUp');
      |         fltRampDown_bkup=get_param(gcb,'fltRampDown');
      |         wf0=Simulink.data.evalinGlobal(bdroot,get_param(gcb,'wf0'));
      |         wksi=Simulink.data.evalinGlobal(bdroot,get_param(gcb,'wksi'));
      |         J=Simulink.data.evalinGlobal(bdroot,get_param(gcb,'J'));
      |         Kt=Simulink.data.evalinGlobal(bdroot,get_param(gcb,'Kt'));
      |         lambdaW=Simulink.data.evalinGlobal(bdroot,get_param(gcb,'lambdaW'));
      |         ramprpm=Simulink.data.evalinGlobal(bdroot,get_param(gcb,'ramprpm'));
      |         mechspeed=Simulink.data.evalinGlobal(bdroot,get_param(gcb,'mechspeed'));
      |         polepairs=Simulink.data.evalinGlobal(bdroot,get_param(gcb,'polepairs'));
      |         if (wf0<=0)
      |           warning('Natural frequency f0 must be positive.');
      |         end
      |         if (wksi<=0)
      |           warning('Current loop attenuation must be positive.');
      |         end
      |         if (wksi>1)
      |           warning('Current loop attenuation must not exceed 1.');
      |         end
      |         if (J<=0)
      |           warning('Moment of inertia J must be positive.');
      |         end
      |         if (Kt<=0)
      |           warning('Torque constant Kt must be positive.');
      |         end
      |         if (lambdaW<0)
      |           warning('MA filter smoothing factor must be in the range 0..1.');
      |         end
      |         if (lambdaW>1)
      |           warning('MA filter smoothing factor must be in the range 0..1.');
      |         end
      |         if (mechspeed<=0)
      |           warning('Max. speed must be positive.');
      |         end
      |         if (polepairs<1)
      |           warning('Number of pole pairs must be a natural number (1, 2, 3, ...).');
      |         end
      |         if (round(polepairs)~=polepairs)
      |           warning('Number of pole pairs must be a natural number (1, 2, 3, ...).');
      |         end
      |         w0=6.283185307179586*wf0;
      |         pgain=2.0*wksi*w0*J/Kt;
      |         igain=w0*w0*J/Kt;
      |         wmax=polepairs*mechspeed*0.1047197551196598;
      |         fltPropGainQ=pgain;
      |         fltIntegGainQ=igain*SampleTime*0.5;
      |         fltLowerLimitQ=-wmax;
      |         fltUpperLimitQ=wmax;
      |         fltLambdaW=lambdaW;
      |         rampsc=polepairs*abs(ramprpm)*0.1047197551196598;
      |         fltRampUp=rampsc;
      |         fltRampDown=rampsc;
      |         if isnan(fltLambdaW)
      |           if ~strcmp(fltLambdaW_bkup,'0')
      |             set_param(gcb,'fltLambdaW','0');
      |           end
      |         else
      |           tmps=num2str(fltLambdaW);
      |           if ~strcmp(fltLambdaW_bkup,tmps)
      |             set_param(gcb,'fltLambdaW',tmps);
      |           end
      |         end
      |         if isnan(fltPropGainQ)
      |           if ~strcmp(fltPropGainQ_bkup,'0')
      |             set_param(gcb,'fltPropGainQ','0');
      |           end
      |         else
      |           tmps=num2str(fltPropGainQ);
      |           if ~strcmp(fltPropGainQ_bkup,tmps)
      |             set_param(gcb,'fltPropGainQ',tmps);
      |           end
      |         end
      |         if isnan(fltIntegGainQ)
      |           if ~strcmp(fltIntegGainQ_bkup,'0')
      |             set_param(gcb,'fltIntegGainQ','0');
      |           end
      |         else
      |           tmps=num2str(fltIntegGainQ);
      |           if ~strcmp(fltIntegGainQ_bkup,tmps)
      |             set_param(gcb,'fltIntegGainQ',tmps);
      |           end
      |         end
      |         if isnan(fltLowerLimitQ)
      |           if ~strcmp(fltLowerLimitQ_bkup,'0')
      |             set_param(gcb,'fltLowerLimitQ','0');
      |           end
      |         else
      |           tmps=num2str(fltLowerLimitQ);
      |           if ~strcmp(fltLowerLimitQ_bkup,tmps)
      |             set_param(gcb,'fltLowerLimitQ',tmps);
      |           end
      |         end
      |         if isnan(fltUpperLimitQ)
      |           if ~strcmp(fltUpperLimitQ_bkup,'0')
      |             set_param(gcb,'fltUpperLimitQ','0');
      |           end
      |         else
      |           tmps=num2str(fltUpperLimitQ);
      |           if ~strcmp(fltUpperLimitQ_bkup,tmps)
      |             set_param(gcb,'fltUpperLimitQ',tmps);
      |           end
      |         end
      |         if isnan(fltRampUp)
      |           if ~strcmp(fltRampUp_bkup,'0')
      |             set_param(gcb,'fltRampUp','0');
      |           end
      |         else
      |           tmps=num2str(fltRampUp);
      |           if ~strcmp(fltRampUp_bkup,tmps)
      |             set_param(gcb,'fltRampUp',tmps);
      |           end
      |         end
      |         if isnan(fltRampDown)
      |           if ~strcmp(fltRampDown_bkup,'0')
      |             set_param(gcb,'fltRampDown','0');
      |           end
      |         else
      |           tmps=num2str(fltRampDown);
      |           if ~strcmp(fltRampDown_bkup,tmps)
      |             set_param(gcb,'fltRampDown',tmps);
      |           end
      |         end
      |       end
      |     end
      |   catch
      |    warning(['Sample time cannot be calculated for the block ' gcb])
      |   end
      | end
      mask DialogControl timeHint Prompt: Note: Implementation parameters cannot be calculated yet because the block's inherited sample time is unknown. Simulink will update the sample time when you run the simulation.
      mask Display:
      | color('black');
      | pos = get_param(gcb, 'Position');
      | width = pos(3) - pos(1);
      | height = pos(4) - pos(2);
      | tX=width/2;
      | tY=height - 25;
      | color('black');
      | text(tX,tY, 'AMCLIB_SpeedLoop_FLT', 'horizontalAlignment', 'center');
      | if showStates == 2
      |   color('red');
      |   text(tX,tY - 20, ['debugging mode' char(13) char(10) '(limited performance)'], 'horizontalAlignment', 'center');
      | end
  AMCLIB_TrackObsrv_FLT : Subsystem  StartFcn=|  TreatAsAtomicUnit=on  mask(AMCLIB_TrackObsrv_FLT){showStates=Hide (faster execution), resetStatesEnable=Pre-set according to the first set of inputs after reset, SampleTime=-1, intmethod=Trapezoidal, if0=350, iksi=1, autoCalcEn=on, fltCC1sc=0, fltCC2sc=0, fltUpperLimit=0, fltLowerLimit=0, fltC1=0, SampleTime_1=NaN}
      | ts=get_param(gcb,'CompiledSampleTime');
      | if iscell(ts)
      |   ts=ts{1};
      |   if iscell(ts)
      |     ts=ts{1};
      |   end
      | end
      | ts=ts(1);
      | set_param(gcb,'SampleTime_1',num2str(ts));
      | p=Simulink.Mask.get(gcb);
      | hintText=p.getDialogControl('timeHint');
      | SampleTime=Simulink.data.evalinGlobal(bdroot,get_param(gcb,'SampleTime'));
      | p=Simulink.Mask.get(gcb);
      | autoCalcEn=get_param(gcb,'autoCalcEn');
      | if strcmp(autoCalcEn,'on')
      |   if SampleTime==-1
      |     hintText.Prompt='Caution: Implementation parameters depend on inherited sample time. Make sure that the sample time of the block''s inputs corresponds to the sampling period in the target application.';
      |   else
      |     hintText.Prompt='Caution: Implementation parameters depend on the sample time. Make sure that the simulation time step corresponds to the sampling period in the target application.';
      |   end
      |   SampleTime=ts;
      |   fltCC1sc_bkup=get_param(gcb,'fltCC1sc');
      |   fltCC2sc_bkup=get_param(gcb,'fltCC2sc');
      |   fltUpperLimit_bkup=get_param(gcb,'fltUpperLimit');
      |   fltLowerLimit_bkup=get_param(gcb,'fltLowerLimit');
      |   fltC1_bkup=get_param(gcb,'fltC1');
      |   intmethod=get_param(gcb,'intmethod');
      |   if0=Simulink.data.evalinGlobal(bdroot,get_param(gcb,'if0'));
      |   iksi=Simulink.data.evalinGlobal(bdroot,get_param(gcb,'iksi'));
      |   if (if0<=0)
      |     warning('Natural frequency f0 must be positive.');
      |   end
      |   if (iksi<=0)
      |     warning('Current loop attenuation must be positive.');
      |   end
      |   if (iksi>1)
      |     warning('Current loop attenuation must not exceed 1.');
      |   end
      |   pgain=12.56637061435917*iksi*if0;
      |   igain=39.47841760435743*if0*if0;
      |   if strcmp(intmethod,'Forward Rectangular')
      |     cc1=pgain;
      |     cc2=-pgain+igain*SampleTime;
      |   else
      |     if strcmp(intmethod,'Backward Rectangular')
      |       cc1=pgain+igain*SampleTime;
      |       cc2=-pgain;
      |     else
      |       cc1=pgain+igain*SampleTime*0.5;
      |       cc2=-pgain+igain*SampleTime*0.5;
      |     end
      |   end
      |   fltCC1sc=cc1;
      |   fltCC2sc=cc2;
      |   fltLowerLimit=-1000000.0;
      |   fltUpperLimit=1000000.0;
      |   fltC1=SampleTime*0.5;
      |   if isnan(fltCC1sc)
      |     if ~strcmp(fltCC1sc_bkup,'0')
      |       set_param(gcb,'fltCC1sc','0');
      |     end
      |   else
      |     tmps=num2str(fltCC1sc);
      |     if ~strcmp(fltCC1sc_bkup,tmps)
      |       set_param(gcb,'fltCC1sc',tmps);
      |     end
      |   end
      |   if isnan(fltCC2sc)
      |     if ~strcmp(fltCC2sc_bkup,'0')
      |       set_param(gcb,'fltCC2sc','0');
      |     end
      |   else
      |     tmps=num2str(fltCC2sc);
      |     if ~strcmp(fltCC2sc_bkup,tmps)
      |       set_param(gcb,'fltCC2sc',tmps);
      |     end
      |   end
      |   if isnan(fltUpperLimit)
      |     if ~strcmp(fltUpperLimit_bkup,'0')
      |       set_param(gcb,'fltUpperLimit','0');
      |     end
      |   else
      |     tmps=num2str(fltUpperLimit);
      |     if ~strcmp(fltUpperLimit_bkup,tmps)
      |       set_param(gcb,'fltUpperLimit',tmps);
      |     end
      |   end
      |   if isnan(fltLowerLimit)
      |     if ~strcmp(fltLowerLimit_bkup,'0')
      |       set_param(gcb,'fltLowerLimit','0');
      |     end
      |   else
      |     tmps=num2str(fltLowerLimit);
      |     if ~strcmp(fltLowerLimit_bkup,tmps)
      |       set_param(gcb,'fltLowerLimit',tmps);
      |     end
      |   end
      |   if isnan(fltC1)
      |     if ~strcmp(fltC1_bkup,'0')
      |       set_param(gcb,'fltC1','0');
      |     end
      |   else
      |     tmps=num2str(fltC1);
      |     if ~strcmp(fltC1_bkup,tmps)
      |       set_param(gcb,'fltC1',tmps);
      |     end
      |   end
      | end
      mask prompts: showStates "Show internal states:"; resetStatesEnable "Internal state after reset:"; SampleTime "Sample time (-1 for inherited):"; intmethod "Integration method:"; if0 "Current loop natural frequency f0 [Hz]:"; iksi "Current loop attenuation ξ:"; autoCalcEn "Calculate implementation parameters from physical parameters"; fltCC1sc "fltCC1sc (GFLIB_ControllerPIrAW - CC1 coefficient):"; fltCC2sc "fltCC2sc (GFLIB_ControllerPIrAW - CC2 coefficient):"; fltUpperLimit "fltUpperLimit (GFLIB_ControllerPIrAW - upper Limit of the controller):"; fltLowerLimit "fltLowerLimit (GFLIB_ControllerPIrAW - lower Limit of the controller):"; fltC1 "fltC1 (GFLIB_IntegratorTR - integrator coefficient):"; SampleTime_1 "Discrete sample time:"
      mask help: Tracking observer in single precision floating-point implementation. This block supports re-initialization of the internal state during simulation. If the block is reset, the outputs of the PI controller and integrator will be aligned with the inputs fltVelocityOut_preset and fltPosOut_preset. The value of fltPosOut_preset must be in the range [-π, π]. Refer to the AMMCLIB User's Guide for further details.
      mask init:
      | ddName = get_param(bdroot,'DataDictionary');
      | if length(ddName)==0
      |   set_param(bdroot,'DataDictionary','ammclib_types.sldd');
      | else
      |   dd = Simulink.data.dictionary.open(ddName);
      |   data = getSection(dd,'Design Data');
      |   if ~exist(data,'SWLIBS_2Syst_F16')
      |     addDataSource(dd,'ammclib_types.sldd');
      |     saveChanges(dd);
      |   end
      | end
      | 
      | if showStates == 1
      |   % hidden state variables
      |   if strcmp(get_param([gcb '/fltCC1'], 'BlockType'), 'Inport')
      |     posblk = get_param(gcb, 'Position');
      | 
      |     pos = get_param([gcb, '/fltCC1'], 'Position');
      |     orient = get_param([gcb, '/fltCC1'], 'Orientation');
      |     delete_block([gcb, '/fltCC1']);
      |     add_block('built-in/Ground', [gcb, '/fltCC1'], 'Position', pos, 'Orientation', orient);
      | 
      |     pos = get_param([gcb, '/fltCC2'], 'Position');
      |     orient = get_param([gcb, '/fltCC2'], 'Orientation');
      |     delete_block([gcb, '/fltCC2']);
      |     add_block('built-in/Ground', [gcb, '/fltCC2'], 'Position', pos, 'Orientation', orient);
      | 
      |     pos = get_param([gcb, '/fltUpperLimit'], 'Position');
      |     orient = get_param([gcb, '/fltUpperLimit'], 'Orientation');
      |     delete_block([gcb, '/fltUpperLimit']);
      |     add_block('built-in/Ground', [gcb, '/fltUpperLimit'], 'Position', pos, 'Orientation', orient);
      | 
      |     pos = get_param([gcb, '/fltLowerLimit'], 'Position');
      |     orient = get_param([gcb, '/fltLowerLimit'], 'Orientation');
      |     delete_block([gcb, '/fltLowerLimit']);
      |     add_block('built-in/Ground', [gcb, '/fltLowerLimit'], 'Position', pos, 'Orientation', orient);
      | 
      |     pos = get_param([gcb, '/fltC1'], 'Position');
      |     orient = get_param([gcb, '/fltC1'], 'Orientation');
      |     delete_block([gcb, '/fltC1']);
      |     add_block('built-in/Ground', [gcb, '/fltC1'], 'Position', pos, 'Orientation', orient);
      | 
      |     pos = get_param([gcb, '/fltAcc'], 'Position');
      |     orient = get_param([gcb, '/fltAcc'], 'Orientation');
      |     delete_block([gcb, '/fltAcc']);
      |     add_block('built-in/Ground', [gcb, '/fltAcc'], 'Position', pos, 'Orientation', orient);
      | 
      |     pos = get_param([gcb, '/fltInErrK1'], 'Position');
      |     orient = get_param([gcb, '/fltInErrK1'], 'Orientation');
      |     delete_block([gcb, '/fltInErrK1']);
      |     add_block('built-in/Ground', [gcb, '/fltInErrK1'], 'Position', pos, 'Orientation', orient);
      | 
      |     pos = get_param([gcb, '/fltState'], 'Position');
      |     orient = get_param([gcb, '/fltState'], 'Orientation');
      |     delete_block([gcb, '/fltState']);
      |     add_block('built-in/Ground', [gcb, '/fltState'], 'Position', pos, 'Orientation', orient);
      | 
      |     pos = get_param([gcb, '/fltInK1'], 'Position');
      |     orient = get_param([gcb, '/fltInK1'], 'Orientation');
      |     delete_block([gcb, '/fltInK1']);
      |     add_block('built-in/Ground', [gcb, '/fltInK1'], 'Position', pos, 'Orientation', orient);
      | 
      | 
      |     pmask=Simulink.Mask.get(gcb);
      |     pctrl=pmask.getParameter('SampleTime');
      |     pctrl.set('TypeOptions',{'fltPhaseErr/SampleTime','fltVelocityOut_preset/SampleTime','fltPosOut_preset/SampleTime'});
      | 
      |     pos = get_param([gcb '/fltAcc_Out'], 'Position');
      |     orient = get_param([gcb '/fltAcc_Out'], 'Orientation');
      |     delete_block([gcb '/fltAcc_Out']);
      |     add_block('built-in/Terminator', [gcb '/fltAcc_Out'], 'Position', pos, 'Orientation', orient);
      | 
      |     pos = get_param([gcb '/fltInErrK1_Out'], 'Position');
      |     orient = get_param([gcb '/fltInErrK1_Out'], 'Orientation');
      |     delete_block([gcb '/fltInErrK1_Out']);
      |     add_block('built-in/Terminator', [gcb '/fltInErrK1_Out'], 'Position', pos, 'Orientation', orient);
      | 
      |     pos = get_param([gcb '/fltState_Out'], 'Position');
      |     orient = get_param([gcb '/fltState_Out'], 'Orientation');
      |     delete_block([gcb '/fltState_Out']);
      |     add_block('built-in/Terminator', [gcb '/fltState_Out'], 'Position', pos, 'Orientation', orient);
      | 
      |     pos = get_param([gcb '/fltInK1_Out'], 'Position');
      |     orient = get_param([gcb '/fltInK1_Out'], 'Orientation');
      |     delete_block([gcb '/fltInK1_Out']);
      |     add_block('built-in/Terminator', [gcb '/fltInK1_Out'], 'Position', pos, 'Orientation', orient);
      | 
      |     set_param([gcb '/fltPhaseErr'], 'Port', '1');
      |     set_param([gcb '/fltVelocityOut_preset'], 'Port', '2');
      |     set_param([gcb '/fltPosOut_preset'], 'Port', '3');
      | 
      |     tmpOutCnt=0;
      |     tmpOutCnt=tmpOutCnt+1;
      |     set_param([gcb '/pPosEst'], 'Port', num2str(tmpOutCnt));
      |     tmpOutCnt=tmpOutCnt+1;
      |     set_param([gcb '/pVelocityEst'], 'Port', num2str(tmpOutCnt));
      | 
      |   autoCalcEn=get_param(gcb,'autoCalcEn');
      |   if strcmp(autoCalcEn,'on')
      |     set_param(gcb,'MaskEnables',{'on','on','on','on','on','on','on','on','on','on','on','on','off'});
      |   else
      |     set_param(gcb,'MaskEnables',{'on','on','on','off','off','off','on','on','on','on','on','on','off'});
      |   end
      | 
      |     if (posblk(4) - posblk(2)) > 100
      |       height = 100;
      |       set_param(gcb,'Position',[posblk(1), posblk(2), posblk(3), posblk(2)+height])
      |     end
      |   end
      | else
      |   % shown state variables
      |   if strcmp(get_param([gcb '/fltCC1'], 'BlockType'), 'Ground')
      |     posblk = get_param(gcb, 'Position');
      | 
      |     pos = get_param([gcb, '/fltCC1'], 'Position');
      |     orient = get_param([gcb, '/fltCC1'], 'Orientation');
      |     delete_block([gcb, '/fltCC1']);
      |     add_block('built-in/Inport', [gcb, '/fltCC1'], 'Position', pos, 'Orientation', orient, 'OutDataTypeStr', 'single');
      | 
      |     pos = get_param([gcb, '/fltCC2'], 'Position');
      |     orient = get_param([gcb, '/fltCC2'], 'Orientation');
      |     delete_block([gcb, '/fltCC2']);
      |     add_block('built-in/Inport', [gcb, '/fltCC2'], 'Position', pos, 'Orientation', orient, 'OutDataTypeStr', 'single');
      | 
      |     pos = get_param([gcb, '/fltUpperLimit'], 'Position');
      |     orient = get_param([gcb, '/fltUpperLimit'], 'Orientation');
      |     delete_block([gcb, '/fltUpperLimit']);
      |     add_block('built-in/Inport', [gcb, '/fltUpperLimit'], 'Position', pos, 'Orientation', orient, 'OutDataTypeStr', 'single');
      | 
      |     pos = get_param([gcb, '/fltLowerLimit'], 'Position');
      |     orient = get_param([gcb, '/fltLowerLimit'], 'Orientation');
      |     delete_block([gcb, '/fltLowerLimit']);
      |     add_block('built-in/Inport', [gcb, '/fltLowerLimit'], 'Position', pos, 'Orientation', orient, 'OutDataTypeStr', 'single');
      | 
      |     pos = get_param([gcb, '/fltC1'], 'Position');
      |     orient = get_param([gcb, '/fltC1'], 'Orientation');
      |     delete_block([gcb, '/fltC1']);
      |     add_block('built-in/Inport', [gcb, '/fltC1'], 'Position', pos, 'Orientation', orient, 'OutDataTypeStr', 'single');
      | 
      |     pos = get_param([gcb, '/fltAcc'], 'Position');
      |     orient = get_param([gcb, '/fltAcc'], 'Orientation');
      |     delete_block([gcb, '/fltAcc']);
      |     add_block('built-in/Inport', [gcb, '/fltAcc'], 'Position', pos, 'Orientation', orient, 'OutDataTypeStr', 'single');
      | 
      |     pos = get_param([gcb, '/fltInErrK1'], 'Position');
      |     orient = get_param([gcb, '/fltInErrK1'], 'Orientation');
      |     delete_block([gcb, '/fltInErrK1']);
      |     add_block('built-in/Inport', [gcb, '/fltInErrK1'], 'Position', pos, 'Orientation', orient, 'OutDataTypeStr', 'single');
      | 
      |     pos = get_param([gcb, '/fltState'], 'Position');
      |     orient = get_param([gcb, '/fltState'], 'Orientation');
      |     delete_block([gcb, '/fltState']);
      |     add_block('built-in/Inport', [gcb, '/fltState'], 'Position', pos, 'Orientation', orient, 'OutDataTypeStr', 'single');
      | 
      |     pos = get_param([gcb, '/fltInK1'], 'Position');
      |     orient = get_param([gcb, '/fltInK1'], 'Orientation');
      |     delete_block([gcb, '/fltInK1']);
      |     add_block('built-in/Inport', [gcb, '/fltInK1'], 'Position', pos, 'Orientation', orient, 'OutDataTypeStr', 'single');
      | 
      | 
      | 
      |     pos = get_param([gcb '/fltAcc_Out'], 'Position');
      |     orient = get_param([gcb '/fltAcc_Out'], 'Orientation');
      |     delete_block([gcb '/fltAcc_Out']);
      |     add_block('built-in/Outport', [gcb '/fltAcc_Out'], 'Position', pos, 'Orientation', orient);
      | 
      |     pos = get_param([gcb '/fltInErrK1_Out'], 'Position');
      |     orient = get_param([gcb '/fltInErrK1_Out'], 'Orientation');
      |     delete_block([gcb '/fltInErrK1_Out']);
      |     add_block('built-in/Outport', [gcb '/fltInErrK1_Out'], 'Position', pos, 'Orientation', orient);
      | 
      |     pos = get_param([gcb '/fltState_Out'], 'Position');
      |     orient = get_param([gcb '/fltState_Out'], 'Orientation');
      |     delete_block([gcb '/fltState_Out']);
      |     add_block('built-in/Outport', [gcb '/fltState_Out'], 'Position', pos, 'Orientation', orient);
      | 
      |     pos = get_param([gcb '/fltInK1_Out'], 'Position');
      |     orient = get_param([gcb '/fltInK1_Out'], 'Orientation');
      |     delete_block([gcb '/fltInK1_Out']);
      |     add_block('built-in/Outport', [gcb '/fltInK1_Out'], 'Position', pos, 'Orientation', orient);
      | 
      | 
      |     pmask=Simulink.Mask.get(gcb);
      |     pctrl=pmask.getParameter('SampleTime');
      |     pctrl.set('TypeOptions',{'fltPhaseErr/SampleTime','fltVelocityOut_preset/SampleTime','fltPosOut_preset/SampleTime','fltCC1/SampleTime','fltCC2/SampleTime','fltUpperLimit/SampleTime','fltLowerLimit/SampleTime','fltC1/SampleTime','fltAcc/SampleTime','fltInErrK1/SampleTime','fltState/SampleTime','fltInK1/SampleTime'});
      | 
      |     set_param([gcb '/fltPhaseErr'], 'Port', '1');
      |     set_param([gcb '/fltVelocityOut_preset'], 'Port', '2');
      |     set_param([gcb '/fltPosOut_preset'], 'Port', '3');
      |     set_param([gcb '/fltCC1'], 'Port', '4');
      |     set_param([gcb '/fltCC2'], 'Port', '5');
      |     set_param([gcb '/fltUpperLimit'], 'Port', '6');
      |     set_param([gcb '/fltLowerLimit'], 'Port', '7');
      |     set_param([gcb '/fltC1'], 'Port', '8');
      |     set_param([gcb '/fltAcc'], 'Port', '9');
      |     set_param([gcb '/fltInErrK1'], 'Port', '10');
      |     set_param([gcb '/fltState'], 'Port', '11');
      |     set_param([gcb '/fltInK1'], 'Port', '12');
      | 
      |     tmpOutCnt=0;
      |     tmpOutCnt=tmpOutCnt+1;
      |     set_param([gcb '/pPosEst'], 'Port', num2str(tmpOutCnt));
      |     tmpOutCnt=tmpOutCnt+1;
      |     set_param([gcb '/pVelocityEst'], 'Port', num2str(tmpOutCnt));
      |     tmpOutCnt=tmpOutCnt+1;
      |     set_param([gcb '/fltAcc_Out'], 'Port', num2str(tmpOutCnt));
      |     tmpOutCnt=tmpOutCnt+1;
      |     set_param([gcb '/fltInErrK1_Out'], 'Port', num2str(tmpOutCnt));
      |     tmpOutCnt=tmpOutCnt+1;
      |     set_param([gcb '/fltState_Out'], 'Port', num2str(tmpOutCnt));
      |     tmpOutCnt=tmpOutCnt+1;
      |     set_param([gcb '/fltInK1_Out'], 'Port', num2str(tmpOutCnt));
      | 
      |     set_param(gcb,'MaskEnables',{'on','on','on','off','off','off','off','off','off','off','off','off','off'});
      | 
      |     if (posblk(4) - posblk(2)) < 325
      |       height = 325;
      |       set_param(gcb,'Position',[posblk(1), posblk(2), posblk(3), posblk(2)+height])
      |     end
      |   end
      | end
      settings: RTWSystemCode=Inline
      mask Help: web([fileparts(which('ammclib_bam_S32K3xx.slx')) '/../doc/S32K3XXMCLUG.pdf'], '-browser')
      mask TypeOptions showStates: Hide (faster execution) | Show (allows debugging; connect feedback loops manually)
      mask Callback showStates:
      | maskStr=get_param(gcb,'showStates');
      | if strcmp(maskStr,'Hide (faster execution)')
      |   autoCalcEn=get_param(gcb,'autoCalcEn');
      |   if strcmp(autoCalcEn,'on')
      |     set_param(gcb,'MaskEnables',{'on','on','on','on','on','on','on','on','on','on','on','on','off'});
      |   else
      |     set_param(gcb,'MaskEnables',{'on','on','on','off','off','off','on','on','on','on','on','on','off'});
      |   end
      | else
      |   set_param(gcb,'MaskEnables',{'on','on','on','off','off','off','off','off','off','off','off','off','off'});
      | end
      mask TypeOptions resetStatesEnable: Pre-set according to the first set of inputs after reset | Clear to zero
      mask TypeOptions SampleTime: fltPhaseErr/SampleTime | fltVelocityOut_preset/SampleTime | fltPosOut_preset/SampleTime
      mask Callback SampleTime:
      | p=Simulink.Mask.get(gcb);
      | hintText=p.getDialogControl('timeHint');
      | SampleTime=Simulink.data.evalinGlobal(bdroot,get_param(gcb,'SampleTime'));
      | SampleTime_1=str2double(get_param(gcb,'SampleTime_1'));
      | if (((SampleTime==-1) && (~contains(hintText.Prompt,'inherited'))) || ...
      |     ((SampleTime~=-1) && contains(hintText.Prompt,'inherited')) || ...
      |     ((SampleTime~=-1) && (SampleTime_1~=SampleTime)) || ...
      |     ((SampleTime_1~=-1) && contains(hintText.Prompt,'yet')))
      |   if ((SampleTime==-1) && (~contains(hintText.Prompt,'inherited')))
      |     set_param(gcb,'SampleTime_1',num2str(NaN));
      |     SampleTime_1=NaN;
      |   end
      |   if (SampleTime~=-1)
      |     set_param(gcb,'SampleTime_1',num2str(SampleTime));
      |     SampleTime_1=SampleTime;
      |   end
      |   autoCalcEn=get_param(gcb,'autoCalcEn');
      |   if strcmp(autoCalcEn,'on')
      |     p=Simulink.Mask.get(gcb);
      |     hintText=p.getDialogControl('timeHint');
      |     if SampleTime==-1
      |       SampleTime=SampleTime_1;
      |       if isnan(SampleTime)
      |         hintText.Prompt='Note: Implementation parameters cannot be calculated yet because the block''s inherited sample time is unknown. Simulink will update the sample time when you run the simulation.';
      |       else
      |         hintText.Prompt='Caution: Implementation parameters depend on inherited sample time. Make sure that the sample time of the block''s inputs corresponds to the sampling period in the target application.';
      |       end
      |     else
      |       hintText.Prompt='Caution: Implementation parameters depend on the sample time. Make sure that the simulation time step corresponds to the sampling period in the target application.';
      |     end
      |     fltCC1sc_bkup=get_param(gcb,'fltCC1sc');
      |     fltCC2sc_bkup=get_param(gcb,'fltCC2sc');
      |     fltUpperLimit_bkup=get_param(gcb,'fltUpperLimit');
      |     fltLowerLimit_bkup=get_param(gcb,'fltLowerLimit');
      |     fltC1_bkup=get_param(gcb,'fltC1');
      |     intmethod=get_param(gcb,'intmethod');
      |     if0=Simulink.data.evalinGlobal(bdroot,get_param(gcb,'if0'));
      |     iksi=Simulink.data.evalinGlobal(bdroot,get_param(gcb,'iksi'));
      |     if (if0<=0)
      |       warning('Natural frequency f0 must be positive.');
      |     end
      |     if (iksi<=0)
      |       warning('Current loop attenuation must be positive.');
      |     end
      |     if (iksi>1)
      |       warning('Current loop attenuation must not exceed 1.');
      |     end
      |     pgain=12.56637061435917*iksi*if0;
      |     igain=39.47841760435743*if0*if0;
      |     if strcmp(intmethod,'Forward Rectangular')
      |       cc1=pgain;
      |       cc2=-pgain+igain*SampleTime;
      |     else
      |       if strcmp(intmethod,'Backward Rectangular')
      |         cc1=pgain+igain*SampleTime;
      |         cc2=-pgain;
      |       else
      |         cc1=pgain+igain*SampleTime*0.5;
      |         cc2=-pgain+igain*SampleTime*0.5;
      |       end
      |     end
      |     fltCC1sc=cc1;
      |     fltCC2sc=cc2;
      |     fltLowerLimit=-1000000.0;
      |     fltUpperLimit=1000000.0;
      |     fltC1=SampleTime*0.5;
      |     if isnan(fltCC1sc)
      |       if ~strcmp(fltCC1sc_bkup,'0')
      |         set_param(gcb,'fltCC1sc','0');
      |       end
      |     else
      |       tmps=num2str(fltCC1sc);
      |       if ~strcmp(fltCC1sc_bkup,tmps)
      |         set_param(gcb,'fltCC1sc',tmps);
      |       end
      |     end
      |     if isnan(fltCC2sc)
      |       if ~strcmp(fltCC2sc_bkup,'0')
      |         set_param(gcb,'fltCC2sc','0');
      |       end
      |     else
      |       tmps=num2str(fltCC2sc);
      |       if ~strcmp(fltCC2sc_bkup,tmps)
      |         set_param(gcb,'fltCC2sc',tmps);
      |       end
      |     end
      |     if isnan(fltUpperLimit)
      |       if ~strcmp(fltUpperLimit_bkup,'0')
      |         set_param(gcb,'fltUpperLimit','0');
      |       end
      |     else
      |       tmps=num2str(fltUpperLimit);
      |       if ~strcmp(fltUpperLimit_bkup,tmps)
      |         set_param(gcb,'fltUpperLimit',tmps);
      |       end
      |     end
      |     if isnan(fltLowerLimit)
      |       if ~strcmp(fltLowerLimit_bkup,'0')
      |         set_param(gcb,'fltLowerLimit','0');
      |       end
      |     else
      |       tmps=num2str(fltLowerLimit);
      |       if ~strcmp(fltLowerLimit_bkup,tmps)
      |         set_param(gcb,'fltLowerLimit',tmps);
      |       end
      |     end
      |     if isnan(fltC1)
      |       if ~strcmp(fltC1_bkup,'0')
      |         set_param(gcb,'fltC1','0');
      |       end
      |     else
      |       tmps=num2str(fltC1);
      |       if ~strcmp(fltC1_bkup,tmps)
      |         set_param(gcb,'fltC1',tmps);
      |       end
      |     end
      |   end
      | end
      mask TypeOptions intmethod: Forward Rectangular | Backward Rectangular | Trapezoidal
      mask Callback intmethod:
      | autoCalcEn=get_param(gcb,'autoCalcEn');
      | if strcmp(autoCalcEn,'on')
      |   SampleTime=Simulink.data.evalinGlobal(bdroot,get_param(gcb,'SampleTime'));
      |   if (SampleTime==-1)
      |     SampleTime=str2double(get_param(gcb,'SampleTime_1'));
      |   end
      |   fltCC1sc_bkup=get_param(gcb,'fltCC1sc');
      |   fltCC2sc_bkup=get_param(gcb,'fltCC2sc');
      |   fltUpperLimit_bkup=get_param(gcb,'fltUpperLimit');
      |   fltLowerLimit_bkup=get_param(gcb,'fltLowerLimit');
      |   fltC1_bkup=get_param(gcb,'fltC1');
      |   intmethod=get_param(gcb,'intmethod');
      |   if0=Simulink.data.evalinGlobal(bdroot,get_param(gcb,'if0'));
      |   iksi=Simulink.data.evalinGlobal(bdroot,get_param(gcb,'iksi'));
      |   if (if0<=0)
      |     warning('Natural frequency f0 must be positive.');
      |   end
      |   if (iksi<=0)
      |     warning('Current loop attenuation must be positive.');
      |   end
      |   if (iksi>1)
      |     warning('Current loop attenuation must not exceed 1.');
      |   end
      |   pgain=12.56637061435917*iksi*if0;
      |   igain=39.47841760435743*if0*if0;
      |   if strcmp(intmethod,'Forward Rectangular')
      |     cc1=pgain;
      |     cc2=-pgain+igain*SampleTime;
      |   else
      |     if strcmp(intmethod,'Backward Rectangular')
      |       cc1=pgain+igain*SampleTime;
      |       cc2=-pgain;
      |     else
      |       cc1=pgain+igain*SampleTime*0.5;
      |       cc2=-pgain+igain*SampleTime*0.5;
      |     end
      |   end
      |   fltCC1sc=cc1;
      |   fltCC2sc=cc2;
      |   fltLowerLimit=-1000000.0;
      |   fltUpperLimit=1000000.0;
      |   fltC1=SampleTime*0.5;
      |   if isnan(fltCC1sc)
      |     if ~strcmp(fltCC1sc_bkup,'0')
      |       set_param(gcb,'fltCC1sc','0');
      |     end
      |   else
      |     tmps=num2str(fltCC1sc);
      |     if ~strcmp(fltCC1sc_bkup,tmps)
      |       set_param(gcb,'fltCC1sc',tmps);
      |     end
      |   end
      |   if isnan(fltCC2sc)
      |     if ~strcmp(fltCC2sc_bkup,'0')
      |       set_param(gcb,'fltCC2sc','0');
      |     end
      |   else
      |     tmps=num2str(fltCC2sc);
      |     if ~strcmp(fltCC2sc_bkup,tmps)
      |       set_param(gcb,'fltCC2sc',tmps);
      |     end
      |   end
      |   if isnan(fltUpperLimit)
      |     if ~strcmp(fltUpperLimit_bkup,'0')
      |       set_param(gcb,'fltUpperLimit','0');
      |     end
      |   else
      |     tmps=num2str(fltUpperLimit);
      |     if ~strcmp(fltUpperLimit_bkup,tmps)
      |       set_param(gcb,'fltUpperLimit',tmps);
      |     end
      |   end
      |   if isnan(fltLowerLimit)
      |     if ~strcmp(fltLowerLimit_bkup,'0')
      |       set_param(gcb,'fltLowerLimit','0');
      |     end
      |   else
      |     tmps=num2str(fltLowerLimit);
      |     if ~strcmp(fltLowerLimit_bkup,tmps)
      |       set_param(gcb,'fltLowerLimit',tmps);
      |     end
      |   end
      |   if isnan(fltC1)
      |     if ~strcmp(fltC1_bkup,'0')
      |       set_param(gcb,'fltC1','0');
      |     end
      |   else
      |     tmps=num2str(fltC1);
      |     if ~strcmp(fltC1_bkup,tmps)
      |       set_param(gcb,'fltC1',tmps);
      |     end
      |   end
      | end
      mask Callback if0:
      | autoCalcEn=get_param(gcb,'autoCalcEn');
      | if strcmp(autoCalcEn,'on')
      |   SampleTime=Simulink.data.evalinGlobal(bdroot,get_param(gcb,'SampleTime'));
      |   if (SampleTime==-1)
      |     SampleTime=str2double(get_param(gcb,'SampleTime_1'));
      |   end
      |   fltCC1sc_bkup=get_param(gcb,'fltCC1sc');
      |   fltCC2sc_bkup=get_param(gcb,'fltCC2sc');
      |   fltUpperLimit_bkup=get_param(gcb,'fltUpperLimit');
      |   fltLowerLimit_bkup=get_param(gcb,'fltLowerLimit');
      |   fltC1_bkup=get_param(gcb,'fltC1');
      |   intmethod=get_param(gcb,'intmethod');
      |   if0=Simulink.data.evalinGlobal(bdroot,get_param(gcb,'if0'));
      |   iksi=Simulink.data.evalinGlobal(bdroot,get_param(gcb,'iksi'));
      |   if (if0<=0)
      |     warning('Natural frequency f0 must be positive.');
      |   end
      |   if (iksi<=0)
      |     warning('Current loop attenuation must be positive.');
      |   end
      |   if (iksi>1)
      |     warning('Current loop attenuation must not exceed 1.');
      |   end
      |   pgain=12.56637061435917*iksi*if0;
      |   igain=39.47841760435743*if0*if0;
      |   if strcmp(intmethod,'Forward Rectangular')
      |     cc1=pgain;
      |     cc2=-pgain+igain*SampleTime;
      |   else
      |     if strcmp(intmethod,'Backward Rectangular')
      |       cc1=pgain+igain*SampleTime;
      |       cc2=-pgain;
      |     else
      |       cc1=pgain+igain*SampleTime*0.5;
      |       cc2=-pgain+igain*SampleTime*0.5;
      |     end
      |   end
      |   fltCC1sc=cc1;
      |   fltCC2sc=cc2;
      |   fltLowerLimit=-1000000.0;
      |   fltUpperLimit=1000000.0;
      |   fltC1=SampleTime*0.5;
      |   if isnan(fltCC1sc)
      |     if ~strcmp(fltCC1sc_bkup,'0')
      |       set_param(gcb,'fltCC1sc','0');
      |     end
      |   else
      |     tmps=num2str(fltCC1sc);
      |     if ~strcmp(fltCC1sc_bkup,tmps)
      |       set_param(gcb,'fltCC1sc',tmps);
      |     end
      |   end
      |   if isnan(fltCC2sc)
      |     if ~strcmp(fltCC2sc_bkup,'0')
      |       set_param(gcb,'fltCC2sc','0');
      |     end
      |   else
      |     tmps=num2str(fltCC2sc);
      |     if ~strcmp(fltCC2sc_bkup,tmps)
      |       set_param(gcb,'fltCC2sc',tmps);
      |     end
      |   end
      |   if isnan(fltUpperLimit)
      |     if ~strcmp(fltUpperLimit_bkup,'0')
      |       set_param(gcb,'fltUpperLimit','0');
      |     end
      |   else
      |     tmps=num2str(fltUpperLimit);
      |     if ~strcmp(fltUpperLimit_bkup,tmps)
      |       set_param(gcb,'fltUpperLimit',tmps);
      |     end
      |   end
      |   if isnan(fltLowerLimit)
      |     if ~strcmp(fltLowerLimit_bkup,'0')
      |       set_param(gcb,'fltLowerLimit','0');
      |     end
      |   else
      |     tmps=num2str(fltLowerLimit);
      |     if ~strcmp(fltLowerLimit_bkup,tmps)
      |       set_param(gcb,'fltLowerLimit',tmps);
      |     end
      |   end
      |   if isnan(fltC1)
      |     if ~strcmp(fltC1_bkup,'0')
      |       set_param(gcb,'fltC1','0');
      |     end
      |   else
      |     tmps=num2str(fltC1);
      |     if ~strcmp(fltC1_bkup,tmps)
      |       set_param(gcb,'fltC1',tmps);
      |     end
      |   end
      | end
      mask Callback iksi:
      | autoCalcEn=get_param(gcb,'autoCalcEn');
      | if strcmp(autoCalcEn,'on')
      |   SampleTime=Simulink.data.evalinGlobal(bdroot,get_param(gcb,'SampleTime'));
      |   if (SampleTime==-1)
      |     SampleTime=str2double(get_param(gcb,'SampleTime_1'));
      |   end
      |   fltCC1sc_bkup=get_param(gcb,'fltCC1sc');
      |   fltCC2sc_bkup=get_param(gcb,'fltCC2sc');
      |   fltUpperLimit_bkup=get_param(gcb,'fltUpperLimit');
      |   fltLowerLimit_bkup=get_param(gcb,'fltLowerLimit');
      |   fltC1_bkup=get_param(gcb,'fltC1');
      |   intmethod=get_param(gcb,'intmethod');
      |   if0=Simulink.data.evalinGlobal(bdroot,get_param(gcb,'if0'));
      |   iksi=Simulink.data.evalinGlobal(bdroot,get_param(gcb,'iksi'));
      |   if (if0<=0)
      |     warning('Natural frequency f0 must be positive.');
      |   end
      |   if (iksi<=0)
      |     warning('Current loop attenuation must be positive.');
      |   end
      |   if (iksi>1)
      |     warning('Current loop attenuation must not exceed 1.');
      |   end
      |   pgain=12.56637061435917*iksi*if0;
      |   igain=39.47841760435743*if0*if0;
      |   if strcmp(intmethod,'Forward Rectangular')
      |     cc1=pgain;
      |     cc2=-pgain+igain*SampleTime;
      |   else
      |     if strcmp(intmethod,'Backward Rectangular')
      |       cc1=pgain+igain*SampleTime;
      |       cc2=-pgain;
      |     else
      |       cc1=pgain+igain*SampleTime*0.5;
      |       cc2=-pgain+igain*SampleTime*0.5;
      |     end
      |   end
      |   fltCC1sc=cc1;
      |   fltCC2sc=cc2;
      |   fltLowerLimit=-1000000.0;
      |   fltUpperLimit=1000000.0;
      |   fltC1=SampleTime*0.5;
      |   if isnan(fltCC1sc)
      |     if ~strcmp(fltCC1sc_bkup,'0')
      |       set_param(gcb,'fltCC1sc','0');
      |     end
      |   else
      |     tmps=num2str(fltCC1sc);
      |     if ~strcmp(fltCC1sc_bkup,tmps)
      |       set_param(gcb,'fltCC1sc',tmps);
      |     end
      |   end
      |   if isnan(fltCC2sc)
      |     if ~strcmp(fltCC2sc_bkup,'0')
      |       set_param(gcb,'fltCC2sc','0');
      |     end
      |   else
      |     tmps=num2str(fltCC2sc);
      |     if ~strcmp(fltCC2sc_bkup,tmps)
      |       set_param(gcb,'fltCC2sc',tmps);
      |     end
      |   end
      |   if isnan(fltUpperLimit)
      |     if ~strcmp(fltUpperLimit_bkup,'0')
      |       set_param(gcb,'fltUpperLimit','0');
      |     end
      |   else
      |     tmps=num2str(fltUpperLimit);
      |     if ~strcmp(fltUpperLimit_bkup,tmps)
      |       set_param(gcb,'fltUpperLimit',tmps);
      |     end
      |   end
      |   if isnan(fltLowerLimit)
      |     if ~strcmp(fltLowerLimit_bkup,'0')
      |       set_param(gcb,'fltLowerLimit','0');
      |     end
      |   else
      |     tmps=num2str(fltLowerLimit);
      |     if ~strcmp(fltLowerLimit_bkup,tmps)
      |       set_param(gcb,'fltLowerLimit',tmps);
      |     end
      |   end
      |   if isnan(fltC1)
      |     if ~strcmp(fltC1_bkup,'0')
      |       set_param(gcb,'fltC1','0');
      |     end
      |   else
      |     tmps=num2str(fltC1);
      |     if ~strcmp(fltC1_bkup,tmps)
      |       set_param(gcb,'fltC1',tmps);
      |     end
      |   end
      | end
      mask Callback autoCalcEn:
      | maskStr=get_param(gcb,'showStates');
      | if strcmp(maskStr,'Hide (faster execution)')
      |   p=Simulink.Mask.get(gcb);
      |   autoCalcEn=get_param(gcb,'autoCalcEn');
      |   hintText=p.getDialogControl('timeHint');
      |   if strcmp(autoCalcEn,'on')
      |     param=p.getParameter('iksi');
      |     if strcmp(param.Enabled,'off')
      |       SampleTime=Simulink.data.evalinGlobal(bdroot,get_param(gcb,'SampleTime'));
      |       if SampleTime==-1
      |         SampleTime=str2double(get_param(gcb,'SampleTime_1'));
      |         if isnan(SampleTime)
      |           hintText.Prompt=['Note: Implementation parameters cannot be calculated yet because the block''s inherited sample time is unknown. Simulink will update the sample time when you run the simulation.'];
      |         else
      |           hintText.Prompt=['Caution: Implementation parameters depend on inherited sample time. Make sure that the sample time of the block''s inputs corresponds to the sampling period in the target application.'];
      |         end
      |       else
      |         hintText.Prompt='Caution: Implementation parameters depend on the sample time. Make sure that the simulation time step corresponds to the sampling period in the target application.';
      |       end
      |       p=Simulink.Mask.get(gcb);
      |       param=p.getParameter('intmethod');
      |       param.set('Enabled','on');
      |       param=p.getParameter('if0');
      |       param.set('Enabled','on');
      |       param=p.getParameter('iksi');
      |       param.set('Enabled','on');
      |     else
      |       SampleTime=Simulink.data.evalinGlobal(bdroot,get_param(gcb,'SampleTime'));
      |       if SampleTime==-1
      |         SampleTime=str2double(get_param(gcb,'SampleTime_1'));
      |       end
      |     end
      |     fltCC1sc_bkup=get_param(gcb,'fltCC1sc');
      |     fltCC2sc_bkup=get_param(gcb,'fltCC2sc');
      |     fltUpperLimit_bkup=get_param(gcb,'fltUpperLimit');
      |     fltLowerLimit_bkup=get_param(gcb,'fltLowerLimit');
      |     fltC1_bkup=get_param(gcb,'fltC1');
      |     intmethod=get_param(gcb,'intmethod');
      |     if0=Simulink.data.evalinGlobal(bdroot,get_param(gcb,'if0'));
      |     iksi=Simulink.data.evalinGlobal(bdroot,get_param(gcb,'iksi'));
      |     if (if0<=0)
      |       warning('Natural frequency f0 must be positive.');
      |     end
      |     if (iksi<=0)
      |       warning('Current loop attenuation must be positive.');
      |     end
      |     if (iksi>1)
      |       warning('Current loop attenuation must not exceed 1.');
      |     end
      |     pgain=12.56637061435917*iksi*if0;
      |     igain=39.47841760435743*if0*if0;
      |     if strcmp(intmethod,'Forward Rectangular')
      |       cc1=pgain;
      |       cc2=-pgain+igain*SampleTime;
      |     else
      |       if strcmp(intmethod,'Backward Rectangular')
      |         cc1=pgain+igain*SampleTime;
      |         cc2=-pgain;
      |       else
      |         cc1=pgain+igain*SampleTime*0.5;
      |         cc2=-pgain+igain*SampleTime*0.5;
      |       end
      |     end
      |     fltCC1sc=cc1;
      |     fltCC2sc=cc2;
      |     fltLowerLimit=-1000000.0;
      |     fltUpperLimit=1000000.0;
      |     fltC1=SampleTime*0.5;
      |     if isnan(fltCC1sc)
      |       if ~strcmp(fltCC1sc_bkup,'0')
      |         set_param(gcb,'fltCC1sc','0');
      |       end
      |     else
      |       tmps=num2str(fltCC1sc);
      |       if ~strcmp(fltCC1sc_bkup,tmps)
      |         set_param(gcb,'fltCC1sc',tmps);
      |       end
      |     end
      |     if isnan(fltCC2sc)
      |       if ~strcmp(fltCC2sc_bkup,'0')
      |         set_param(gcb,'fltCC2sc','0');
      |       end
      |     else
      |       tmps=num2str(fltCC2sc);
      |       if ~strcmp(fltCC2sc_bkup,tmps)
      |         set_param(gcb,'fltCC2sc',tmps);
      |       end
      |     end
      |     if isnan(fltUpperLimit)
      |       if ~strcmp(fltUpperLimit_bkup,'0')
      |         set_param(gcb,'fltUpperLimit','0');
      |       end
      |     else
      |       tmps=num2str(fltUpperLimit);
      |       if ~strcmp(fltUpperLimit_bkup,tmps)
      |         set_param(gcb,'fltUpperLimit',tmps);
      |       end
      |     end
      |     if isnan(fltLowerLimit)
      |       if ~strcmp(fltLowerLimit_bkup,'0')
      |         set_param(gcb,'fltLowerLimit','0');
      |       end
      |     else
      |       tmps=num2str(fltLowerLimit);
      |       if ~strcmp(fltLowerLimit_bkup,tmps)
      |         set_param(gcb,'fltLowerLimit',tmps);
      |       end
      |     end
      |     if isnan(fltC1)
      |       if ~strcmp(fltC1_bkup,'0')
      |         set_param(gcb,'fltC1','0');
      |       end
      |     else
      |       tmps=num2str(fltC1);
      |       if ~strcmp(fltC1_bkup,tmps)
      |         set_param(gcb,'fltC1',tmps);
      |       end
      |     end
      |   else
      |     param=p.getParameter('iksi');
      |     if strcmp(param.Enabled,'on')
      |       hintText.Prompt='Caution: Implementation parameters are fixed.';
      |       p=Simulink.Mask.get(gcb);
      |       param=p.getParameter('intmethod');
      |       param.set('Enabled','off');
      |       param=p.getParameter('if0');
      |       param.set('Enabled','off');
      |       param=p.getParameter('iksi');
      |       param.set('Enabled','off');
      |     end
      |   end
      | end
      mask DialogControl CompBut Prompt: Recalculate sample times
      mask DialogControl CompBut Tooltip: Simulink updates the sample times of all blocks when the simulation is run. This button will update the sample times now.
      mask DialogControl CompBut Callback:
      | btn=questdlg('This will apply all changes in all open dialog boxes and update the schematic. Do you want to proceed?','Apply all changes','Continue','Cancel','Continue');
      | if strcmp(btn,'Continue')
      |   dlgs=DAStudio.ToolRoot.getOpenDialogs;
      |   for i=1:length(dlgs)
      |     dlgs(i).apply;
      |   end
      |   try
      |     SampleTime_1=str2double(get_param(gcb,'SampleTime_1'));
      |     ts=Simulink.Block.getSampleTimes(gcb);
      |     ts=ts(1).Value(1);
      |     if (SampleTime_1 ~= ts)
      |       SampleTime_1=ts;
      |       set_param(gcb,'SampleTime_1',num2str(ts));
      |       autoCalcEn=get_param(gcb,'autoCalcEn');
      |       if strcmp(autoCalcEn,'on')
      |         SampleTime=Simulink.data.evalinGlobal(bdroot,get_param(gcb,'SampleTime'));
      |         p=Simulink.Mask.get(gcb);
      |         hintText=p.getDialogControl('timeHint');
      |         if SampleTime==-1
      |           SampleTime=SampleTime_1;
      |           hintText.Prompt='Caution: Implementation parameters depend on inherited sample time. Make sure that the sample time of the block''s inputs corresponds to the sampling period in the target application.';
      |         else
      |           hintText.Prompt='Caution: Implementation parameters depend on the sample time. Make sure that the simulation time step corresponds to the sampling period in the target application.';
      |         end
      |         fltCC1sc_bkup=get_param(gcb,'fltCC1sc');
      |         fltCC2sc_bkup=get_param(gcb,'fltCC2sc');
      |         fltUpperLimit_bkup=get_param(gcb,'fltUpperLimit');
      |         fltLowerLimit_bkup=get_param(gcb,'fltLowerLimit');
      |         fltC1_bkup=get_param(gcb,'fltC1');
      |         intmethod=get_param(gcb,'intmethod');
      |         if0=Simulink.data.evalinGlobal(bdroot,get_param(gcb,'if0'));
      |         iksi=Simulink.data.evalinGlobal(bdroot,get_param(gcb,'iksi'));
      |         if (if0<=0)
